simulink model "model"  (R2014a)
(part 4 of 5)

      | %<Name>
  bus355 : powerlib/Measurements/Load Flow Bus  LConnTagsString=a  ID=bus355  Vbase=110000  Vref=1  Vangle=0  VLF=1  angleLF=0
      settings: AttributesFormatString=|
      | %<ID>
      | %<Vbase>V
      | %<VLF>pu
      | %<angleLF>deg.
      | %<Name>
  bus356 : powerlib/Measurements/Load Flow Bus  LConnTagsString=a  ID=bus356  Vbase=220000  Vref=1  Vangle=0  VLF=1  angleLF=0
      settings: AttributesFormatString=|
      | %<ID>
      | %<Vbase>V
      | %<VLF>pu
      | %<angleLF>deg.
      | %<Name>
  bus357 : powerlib/Measurements/Load Flow Bus  LConnTagsString=a  ID=bus357  Vbase=220000  Vref=1  Vangle=0  VLF=1  angleLF=0
      settings: AttributesFormatString=|
      | %<ID>
      | %<Vbase>V
      | %<VLF>pu
      | %<angleLF>deg.
      | %<Name>
  bus358 : powerlib/Measurements/Load Flow Bus  LConnTagsString=a  ID=bus358  Vbase=220000  Vref=1  Vangle=0  VLF=1  angleLF=0
      settings: AttributesFormatString=|
      | %<ID>
      | %<Vbase>V
      | %<VLF>pu
      | %<angleLF>deg.
      | %<Name>
  bus359 : powerlib/Measurements/Load Flow Bus  LConnTagsString=a  ID=bus359  Vbase=220000  Vref=1  Vangle=0  VLF=1  angleLF=0
      settings: AttributesFormatString=|
      | %<ID>
      | %<Vbase>V
      | %<VLF>pu
      | %<angleLF>deg.
      | %<Name>
  bus36 : powerlib/Measurements/Load Flow Bus  LConnTagsString=a  ID=bus36  Vbase=220000  Vref=1  Vangle=0  VLF=1  angleLF=0
      settings: AttributesFormatString=|
      | %<ID>
      | %<Vbase>V
      | %<VLF>pu
      | %<angleLF>deg.
      | %<Name>
  bus360 : powerlib/Measurements/Load Flow Bus  LConnTagsString=a  ID=bus360  Vbase=220000  Vref=1  Vangle=0  VLF=1  angleLF=0
      settings: AttributesFormatString=|
      | %<ID>
      | %<Vbase>V
      | %<VLF>pu
      | %<angleLF>deg.
      | %<Name>
  bus361 : powerlib/Measurements/Load Flow Bus  LConnTagsString=a  ID=bus361  Vbase=220000  Vref=1  Vangle=0  VLF=1  angleLF=0
      settings: AttributesFormatString=|
      | %<ID>
      | %<Vbase>V
      | %<VLF>pu
      | %<angleLF>deg.
      | %<Name>
  bus362 : powerlib/Measurements/Load Flow Bus  LConnTagsString=a  ID=bus362  Vbase=220000  Vref=1  Vangle=0  VLF=1  angleLF=0
      settings: AttributesFormatString=|
      | %<ID>
      | %<Vbase>V
      | %<VLF>pu
      | %<angleLF>deg.
      | %<Name>
  bus363 : powerlib/Measurements/Load Flow Bus  LConnTagsString=a  ID=bus363  Vbase=220000  Vref=1  Vangle=0  VLF=1  angleLF=0
      settings: AttributesFormatString=|
      | %<ID>
      | %<Vbase>V
      | %<VLF>pu
      | %<angleLF>deg.
      | %<Name>
  bus364 : powerlib/Measurements/Load Flow Bus  LConnTagsString=a  ID=bus364  Vbase=220000  Vref=1  Vangle=0  VLF=1  angleLF=0
      settings: AttributesFormatString=|
      | %<ID>
      | %<Vbase>V
      | %<VLF>pu
      | %<angleLF>deg.
      | %<Name>
  bus365 : powerlib/Measurements/Load Flow Bus  LConnTagsString=a  ID=bus365  Vbase=220000  Vref=1  Vangle=0  VLF=1  angleLF=0
      settings: AttributesFormatString=|
      | %<ID>
      | %<Vbase>V
      | %<VLF>pu
      | %<angleLF>deg.
      | %<Name>
  bus366 : powerlib/Measurements/Load Flow Bus  LConnTagsString=a  ID=bus366  Vbase=220000  Vref=1  Vangle=0  VLF=1  angleLF=0
      settings: AttributesFormatString=|
      | %<ID>
      | %<Vbase>V
      | %<VLF>pu
      | %<angleLF>deg.
      | %<Name>
  bus367 : powerlib/Measurements/Load Flow Bus  LConnTagsString=a  ID=bus367  Vbase=220000  Vref=1  Vangle=0  VLF=1  angleLF=0
      settings: AttributesFormatString=|
      | %<ID>
      | %<Vbase>V
      | %<VLF>pu
      | %<angleLF>deg.
      | %<Name>
  bus368 : powerlib/Measurements/Load Flow Bus  LConnTagsString=a  ID=bus368  Vbase=220000  Vref=1  Vangle=0  VLF=1  angleLF=0
      settings: AttributesFormatString=|
      | %<ID>
      | %<Vbase>V
      | %<VLF>pu
      | %<angleLF>deg.
      | %<Name>
  bus369 : powerlib/Measurements/Load Flow Bus  LConnTagsString=a  ID=bus369  Vbase=220000  Vref=1  Vangle=0  VLF=1  angleLF=0
      settings: AttributesFormatString=|
      | %<ID>
      | %<Vbase>V
      | %<VLF>pu
      | %<angleLF>deg.
      | %<Name>
  bus37 : powerlib/Measurements/Load Flow Bus  LConnTagsString=a  ID=bus37  Vbase=220000  Vref=1  Vangle=0  VLF=1  angleLF=0
      settings: AttributesFormatString=|
      | %<ID>
      | %<Vbase>V
      | %<VLF>pu
      | %<angleLF>deg.
      | %<Name>
  bus370 : powerlib/Measurements/Load Flow Bus  LConnTagsString=a  ID=bus370  Vbase=220000  Vref=1  Vangle=0  VLF=1  angleLF=0
      settings: AttributesFormatString=|
      | %<ID>
      | %<Vbase>V
      | %<VLF>pu
      | %<angleLF>deg.
      | %<Name>
  bus371 : powerlib/Measurements/Load Flow Bus  LConnTagsString=a  ID=bus371  Vbase=220000  Vref=1  Vangle=0  VLF=1  angleLF=0
      settings: AttributesFormatString=|
      | %<ID>
      | %<Vbase>V
      | %<VLF>pu
      | %<angleLF>deg.
      | %<Name>
  bus372 : powerlib/Measurements/Load Flow Bus  LConnTagsString=a  ID=bus372  Vbase=220000  Vref=1  Vangle=0  VLF=1  angleLF=0
      settings: AttributesFormatString=|
      | %<ID>
      | %<Vbase>V
      | %<VLF>pu
      | %<angleLF>deg.
      | %<Name>
  bus373 : powerlib/Measurements/Load Flow Bus  LConnTagsString=a  ID=bus373  Vbase=220000  Vref=1  Vangle=0  VLF=1  angleLF=0
      settings: AttributesFormatString=|
      | %<ID>
      | %<Vbase>V
      | %<VLF>pu
      | %<angleLF>deg.
      | %<Name>
  bus374 : powerlib/Measurements/Load Flow Bus  LConnTagsString=a  ID=bus374  Vbase=220000  Vref=1  Vangle=0  VLF=1  angleLF=0
      settings: AttributesFormatString=|
      | %<ID>
      | %<Vbase>V
      | %<VLF>pu
      | %<angleLF>deg.
      | %<Name>
  bus375 : powerlib/Measurements/Load Flow Bus  LConnTagsString=a  ID=bus375  Vbase=220000  Vref=1  Vangle=0  VLF=1  angleLF=0
      settings: AttributesFormatString=|
      | %<ID>
      | %<Vbase>V
      | %<VLF>pu
      | %<angleLF>deg.
      | %<Name>
  bus376 : powerlib/Measurements/Load Flow Bus  LConnTagsString=a  ID=bus376  Vbase=220000  Vref=1  Vangle=0  VLF=1  angleLF=0
      settings: AttributesFormatString=|
      | %<ID>
      | %<Vbase>V
      | %<VLF>pu
      | %<angleLF>deg.
      | %<Name>
  bus377 : powerlib/Measurements/Load Flow Bus  LConnTagsString=a  ID=bus377  Vbase=220000  Vref=1  Vangle=0  VLF=1  angleLF=0
      settings: AttributesFormatString=|
      | %<ID>
      | %<Vbase>V
      | %<VLF>pu
      | %<angleLF>deg.
      | %<Name>
  bus378 : powerlib/Measurements/Load Flow Bus  LConnTagsString=a  ID=bus378  Vbase=220000  Vref=1  Vangle=0  VLF=1  angleLF=0
      settings: AttributesFormatString=|
      | %<ID>
      | %<Vbase>V
      | %<VLF>pu
      | %<angleLF>deg.
      | %<Name>
  bus379 : powerlib/Measurements/Load Flow Bus  LConnTagsString=a  ID=bus379  Vbase=220000  Vref=1  Vangle=0  VLF=1  angleLF=0
      settings: AttributesFormatString=|
      | %<ID>
      | %<Vbase>V
      | %<VLF>pu
      | %<angleLF>deg.
      | %<Name>
  bus38 : powerlib/Measurements/Load Flow Bus  LConnTagsString=a  ID=bus38  Vbase=220000  Vref=1  Vangle=0  VLF=1  angleLF=0
      settings: AttributesFormatString=|
      | %<ID>
      | %<Vbase>V
      | %<VLF>pu
      | %<angleLF>deg.
      | %<Name>
  bus380 : powerlib/Measurements/Load Flow Bus  LConnTagsString=a  ID=bus380  Vbase=220000  Vref=1  Vangle=0  VLF=1  angleLF=0
      settings: AttributesFormatString=|
      | %<ID>
      | %<Vbase>V
      | %<VLF>pu
      | %<angleLF>deg.
      | %<Name>
  bus381 : powerlib/Measurements/Load Flow Bus  LConnTagsString=a  ID=bus381  Vbase=220000  Vref=1  Vangle=0  VLF=1  angleLF=0
      settings: AttributesFormatString=|
      | %<ID>
      | %<Vbase>V
      | %<VLF>pu
      | %<angleLF>deg.
      | %<Name>
  bus382 : powerlib/Measurements/Load Flow Bus  LConnTagsString=a  ID=bus382  Vbase=220000  Vref=1  Vangle=0  VLF=1  angleLF=0
      settings: AttributesFormatString=|
      | %<ID>
      | %<Vbase>V
      | %<VLF>pu
      | %<angleLF>deg.
      | %<Name>
  bus383 : powerlib/Measurements/Load Flow Bus  LConnTagsString=a  ID=bus383  Vbase=220000  Vref=1  Vangle=0  VLF=1  angleLF=0
      settings: AttributesFormatString=|
      | %<ID>
      | %<Vbase>V
      | %<VLF>pu
      | %<angleLF>deg.
      | %<Name>
  bus384 : powerlib/Measurements/Load Flow Bus  LConnTagsString=a  ID=bus384  Vbase=220000  Vref=1  Vangle=0  VLF=1  angleLF=0
      settings: AttributesFormatString=|
      | %<ID>
      | %<Vbase>V
      | %<VLF>pu
      | %<angleLF>deg.
      | %<Name>
  bus385 : powerlib/Measurements/Load Flow Bus  LConnTagsString=a  ID=bus385  Vbase=220000  Vref=1  Vangle=0  VLF=1  angleLF=0
      settings: AttributesFormatString=|
      | %<ID>
      | %<Vbase>V
      | %<VLF>pu
      | %<angleLF>deg.
      | %<Name>
  bus386 : powerlib/Measurements/Load Flow Bus  LConnTagsString=a  ID=bus386  Vbase=220000  Vref=1  Vangle=0  VLF=1  angleLF=0
      settings: AttributesFormatString=|
      | %<ID>
      | %<Vbase>V
      | %<VLF>pu
      | %<angleLF>deg.
      | %<Name>
  bus387 : powerlib/Measurements/Load Flow Bus  LConnTagsString=a  ID=bus387  Vbase=220000  Vref=1  Vangle=0  VLF=1  angleLF=0
      settings: AttributesFormatString=|
      | %<ID>
      | %<Vbase>V
      | %<VLF>pu
      | %<angleLF>deg.
      | %<Name>
  bus388 : powerlib/Measurements/Load Flow Bus  LConnTagsString=a  ID=bus388  Vbase=220000  Vref=1  Vangle=0  VLF=1  angleLF=0
      settings: AttributesFormatString=|
      | %<ID>
      | %<Vbase>V
      | %<VLF>pu
      | %<angleLF>deg.
      | %<Name>
  bus389 : powerlib/Measurements/Load Flow Bus  LConnTagsString=a  ID=bus389  Vbase=220000  Vref=1  Vangle=0  VLF=1  angleLF=0
      settings: AttributesFormatString=|
      | %<ID>
      | %<Vbase>V
      | %<VLF>pu
      | %<angleLF>deg.
      | %<Name>
  bus39 : powerlib/Measurements/Load Flow Bus  LConnTagsString=a  ID=bus39  Vbase=220000  Vref=1  Vangle=0  VLF=1  angleLF=0
      settings: AttributesFormatString=|
      | %<ID>
      | %<Vbase>V
      | %<VLF>pu
      | %<angleLF>deg.
      | %<Name>
  bus390 : powerlib/Measurements/Load Flow Bus  LConnTagsString=a  ID=bus390  Vbase=220000  Vref=1  Vangle=0  VLF=1  angleLF=0
      settings: AttributesFormatString=|
      | %<ID>
      | %<Vbase>V
      | %<VLF>pu
      | %<angleLF>deg.
      | %<Name>
  bus391 : powerlib/Measurements/Load Flow Bus  LConnTagsString=a  ID=bus391  Vbase=220000  Vref=1  Vangle=0  VLF=1  angleLF=0
      settings: AttributesFormatString=|
      | %<ID>
      | %<Vbase>V
      | %<VLF>pu
      | %<angleLF>deg.
      | %<Name>
  bus392 : powerlib/Measurements/Load Flow Bus  LConnTagsString=a  ID=bus392  Vbase=220000  Vref=1  Vangle=0  VLF=1  angleLF=0
      settings: AttributesFormatString=|
      | %<ID>
      | %<Vbase>V
      | %<VLF>pu
      | %<angleLF>deg.
      | %<Name>
  bus393 : powerlib/Measurements/Load Flow Bus  LConnTagsString=a  ID=bus393  Vbase=220000  Vref=1  Vangle=0  VLF=1  angleLF=0
      settings: AttributesFormatString=|
      | %<ID>
      | %<Vbase>V
      | %<VLF>pu
      | %<angleLF>deg.
      | %<Name>
  bus394 : powerlib/Measurements/Load Flow Bus  LConnTagsString=a  ID=bus394  Vbase=220000  Vref=1  Vangle=0  VLF=1  angleLF=0
      settings: AttributesFormatString=|
      | %<ID>
      | %<Vbase>V
      | %<VLF>pu
      | %<angleLF>deg.
      | %<Name>
  bus395 : powerlib/Measurements/Load Flow Bus  LConnTagsString=a  ID=bus395  Vbase=220000  Vref=1  Vangle=0  VLF=1  angleLF=0
      settings: AttributesFormatString=|
      | %<ID>
      | %<Vbase>V
      | %<VLF>pu
      | %<angleLF>deg.
      | %<Name>
  bus396 : powerlib/Measurements/Load Flow Bus  LConnTagsString=a  ID=bus396  Vbase=220000  Vref=1  Vangle=0  VLF=1  angleLF=0
      settings: AttributesFormatString=|
      | %<ID>
      | %<Vbase>V
      | %<VLF>pu
      | %<angleLF>deg.
      | %<Name>
  bus397 : powerlib/Measurements/Load Flow Bus  LConnTagsString=a  ID=bus397  Vbase=220000  Vref=1  Vangle=0  VLF=1  angleLF=0
      settings: AttributesFormatString=|
      | %<ID>
      | %<Vbase>V
      | %<VLF>pu
      | %<angleLF>deg.
      | %<Name>
  bus398 : powerlib/Measurements/Load Flow Bus  LConnTagsString=a  ID=bus398  Vbase=220000  Vref=1  Vangle=0  VLF=1  angleLF=0
      settings: AttributesFormatString=|
      | %<ID>
      | %<Vbase>V
      | %<VLF>pu
      | %<angleLF>deg.
      | %<Name>
  bus399 : powerlib/Measurements/Load Flow Bus  LConnTagsString=a  ID=bus399  Vbase=220000  Vref=1  Vangle=0  VLF=1  angleLF=0
      settings: AttributesFormatString=|
      | %<ID>
      | %<Vbase>V
      | %<VLF>pu
      | %<angleLF>deg.
      | %<Name>
  bus4 : powerlib/Measurements/Load Flow Bus  LConnTagsString=a  ID=bus4  Vbase=110000  Vref=1  Vangle=0  VLF=1  angleLF=0
      settings: AttributesFormatString=|
      | %<ID>
      | %<Vbase>V
      | %<VLF>pu
      | %<angleLF>deg.
      | %<Name>
  bus40 : powerlib/Measurements/Load Flow Bus  LConnTagsString=a  ID=bus40  Vbase=220000  Vref=1  Vangle=0  VLF=1  angleLF=0
      settings: AttributesFormatString=|
      | %<ID>
      | %<Vbase>V
      | %<VLF>pu
      | %<angleLF>deg.
      | %<Name>
  bus400 : powerlib/Measurements/Load Flow Bus  LConnTagsString=a  ID=bus400  Vbase=220000  Vref=1  Vangle=0  VLF=1  angleLF=0
      settings: AttributesFormatString=|
      | %<ID>
      | %<Vbase>V
      | %<VLF>pu
      | %<angleLF>deg.
      | %<Name>
  bus401 : powerlib/Measurements/Load Flow Bus  LConnTagsString=a  ID=bus401  Vbase=220000  Vref=1  Vangle=0  VLF=1  angleLF=0
      settings: AttributesFormatString=|
      | %<ID>
      | %<Vbase>V
      | %<VLF>pu
      | %<angleLF>deg.
      | %<Name>
  bus402 : powerlib/Measurements/Load Flow Bus  LConnTagsString=a  ID=bus402  Vbase=220000  Vref=1  Vangle=0  VLF=1  angleLF=0
      settings: AttributesFormatString=|
      | %<ID>
      | %<Vbase>V
      | %<VLF>pu
      | %<angleLF>deg.
      | %<Name>
  bus403 : powerlib/Measurements/Load Flow Bus  LConnTagsString=a  ID=bus403  Vbase=220000  Vref=1  Vangle=0  VLF=1  angleLF=0
      settings: AttributesFormatString=|
      | %<ID>
      | %<Vbase>V
      | %<VLF>pu
      | %<angleLF>deg.
      | %<Name>
  bus404 : powerlib/Measurements/Load Flow Bus  LConnTagsString=a  ID=bus404  Vbase=220000  Vref=1  Vangle=0  VLF=1  angleLF=0
      settings: AttributesFormatString=|
      | %<ID>
      | %<Vbase>V
      | %<VLF>pu
      | %<angleLF>deg.
      | %<Name>
  bus405 : powerlib/Measurements/Load Flow Bus  LConnTagsString=a  ID=bus405  Vbase=220000  Vref=1  Vangle=0  VLF=1  angleLF=0
      settings: AttributesFormatString=|
      | %<ID>
      | %<Vbase>V
      | %<VLF>pu
      | %<angleLF>deg.
      | %<Name>
  bus406 : powerlib/Measurements/Load Flow Bus  LConnTagsString=a  ID=bus406  Vbase=220000  Vref=1  Vangle=0  VLF=1  angleLF=0
      settings: AttributesFormatString=|
      | %<ID>
      | %<Vbase>V
      | %<VLF>pu
      | %<angleLF>deg.
      | %<Name>
  bus407 : powerlib/Measurements/Load Flow Bus  LConnTagsString=a  ID=bus407  Vbase=220000  Vref=1  Vangle=0  VLF=1  angleLF=0
      settings: AttributesFormatString=|
      | %<ID>
      | %<Vbase>V
      | %<VLF>pu
      | %<angleLF>deg.
      | %<Name>
  bus408 : powerlib/Measurements/Load Flow Bus  LConnTagsString=a  ID=bus408  Vbase=220000  Vref=1  Vangle=0  VLF=1  angleLF=0
      settings: AttributesFormatString=|
      | %<ID>
      | %<Vbase>V
      | %<VLF>pu
      | %<angleLF>deg.
      | %<Name>
  bus409 : powerlib/Measurements/Load Flow Bus  LConnTagsString=a  ID=bus409  Vbase=220000  Vref=1  Vangle=0  VLF=1  angleLF=0
      settings: AttributesFormatString=|
      | %<ID>
      | %<Vbase>V
      | %<VLF>pu
      | %<angleLF>deg.
      | %<Name>
  bus41 : powerlib/Measurements/Load Flow Bus  LConnTagsString=a  ID=bus41  Vbase=220000  Vref=1  Vangle=0  VLF=1  angleLF=0
      settings: AttributesFormatString=|
      | %<ID>
      | %<Vbase>V
      | %<VLF>pu
      | %<angleLF>deg.
      | %<Name>
  bus410 : powerlib/Measurements/Load Flow Bus  LConnTagsString=a  ID=bus410  Vbase=220000  Vref=1  Vangle=0  VLF=1  angleLF=0
      settings: AttributesFormatString=|
      | %<ID>
      | %<Vbase>V
      | %<VLF>pu
      | %<angleLF>deg.
      | %<Name>
  bus411 : powerlib/Measurements/Load Flow Bus  LConnTagsString=a  ID=bus411  Vbase=220000  Vref=1  Vangle=0  VLF=1  angleLF=0
      settings: AttributesFormatString=|
      | %<ID>
      | %<Vbase>V
      | %<VLF>pu
      | %<angleLF>deg.
      | %<Name>
  bus412 : powerlib/Measurements/Load Flow Bus  LConnTagsString=a  ID=bus412  Vbase=220000  Vref=1  Vangle=0  VLF=1  angleLF=0
      settings: AttributesFormatString=|
      | %<ID>
      | %<Vbase>V
      | %<VLF>pu
      | %<angleLF>deg.
      | %<Name>
  bus413 : powerlib/Measurements/Load Flow Bus  LConnTagsString=a  ID=bus413  Vbase=220000  Vref=1  Vangle=0  VLF=1  angleLF=0
      settings: AttributesFormatString=|
      | %<ID>
      | %<Vbase>V
      | %<VLF>pu
      | %<angleLF>deg.
      | %<Name>
  bus414 : powerlib/Measurements/Load Flow Bus  LConnTagsString=a  ID=bus414  Vbase=220000  Vref=1  Vangle=0  VLF=1  angleLF=0
      settings: AttributesFormatString=|
      | %<ID>
      | %<Vbase>V
      | %<VLF>pu
      | %<angleLF>deg.
      | %<Name>
  bus415 : powerlib/Measurements/Load Flow Bus  LConnTagsString=a  ID=bus415  Vbase=220000  Vref=1  Vangle=0  VLF=1  angleLF=0
      settings: AttributesFormatString=|
      | %<ID>
      | %<Vbase>V
      | %<VLF>pu
      | %<angleLF>deg.
      | %<Name>
  bus416 : powerlib/Measurements/Load Flow Bus  LConnTagsString=a  ID=bus416  Vbase=220000  Vref=1  Vangle=0  VLF=1  angleLF=0
      settings: AttributesFormatString=|
      | %<ID>
      | %<Vbase>V
      | %<VLF>pu
      | %<angleLF>deg.
      | %<Name>
  bus417 : powerlib/Measurements/Load Flow Bus  LConnTagsString=a  ID=bus417  Vbase=220000  Vref=1  Vangle=0  VLF=1  angleLF=0
      settings: AttributesFormatString=|
      | %<ID>
      | %<Vbase>V
      | %<VLF>pu
      | %<angleLF>deg.
      | %<Name>
  bus418 : powerlib/Measurements/Load Flow Bus  LConnTagsString=a  ID=bus418  Vbase=220000  Vref=1  Vangle=0  VLF=1  angleLF=0
      settings: AttributesFormatString=|
      | %<ID>
      | %<Vbase>V
      | %<VLF>pu
      | %<angleLF>deg.
      | %<Name>
  bus419 : powerlib/Measurements/Load Flow Bus  LConnTagsString=a  ID=bus419  Vbase=220000  Vref=1  Vangle=0  VLF=1  angleLF=0
      settings: AttributesFormatString=|
      | %<ID>
      | %<Vbase>V
      | %<VLF>pu
      | %<angleLF>deg.
      | %<Name>
  bus42 : powerlib/Measurements/Load Flow Bus  LConnTagsString=a  ID=bus42  Vbase=220000  Vref=1  Vangle=0  VLF=1  angleLF=0
      settings: AttributesFormatString=|
      | %<ID>
      | %<Vbase>V
      | %<VLF>pu
      | %<angleLF>deg.
      | %<Name>
  bus420 : powerlib/Measurements/Load Flow Bus  LConnTagsString=a  ID=bus420  Vbase=220000  Vref=1  Vangle=0  VLF=1  angleLF=0
      settings: AttributesFormatString=|
      | %<ID>
      | %<Vbase>V
      | %<VLF>pu
      | %<angleLF>deg.
      | %<Name>
  bus421 : powerlib/Measurements/Load Flow Bus  LConnTagsString=a  ID=bus421  Vbase=220000  Vref=1  Vangle=0  VLF=1  angleLF=0
      settings: AttributesFormatString=|
      | %<ID>
      | %<Vbase>V
      | %<VLF>pu
      | %<angleLF>deg.
      | %<Name>
  bus422 : powerlib/Measurements/Load Flow Bus  LConnTagsString=a  ID=bus422  Vbase=220000  Vref=1  Vangle=0  VLF=1  angleLF=0
      settings: AttributesFormatString=|
      | %<ID>
      | %<Vbase>V
      | %<VLF>pu
      | %<angleLF>deg.
      | %<Name>
  bus423 : powerlib/Measurements/Load Flow Bus  LConnTagsString=a  ID=bus423  Vbase=220000  Vref=1  Vangle=0  VLF=1  angleLF=0
      settings: AttributesFormatString=|
      | %<ID>
      | %<Vbase>V
      | %<VLF>pu
      | %<angleLF>deg.
      | %<Name>
  bus424 : powerlib/Measurements/Load Flow Bus  LConnTagsString=a  ID=bus424  Vbase=220000  Vref=1  Vangle=0  VLF=1  angleLF=0
      settings: AttributesFormatString=|
      | %<ID>
      | %<Vbase>V
      | %<VLF>pu
      | %<angleLF>deg.
      | %<Name>
  bus425 : powerlib/Measurements/Load Flow Bus  LConnTagsString=a  ID=bus425  Vbase=220000  Vref=1  Vangle=0  VLF=1  angleLF=0
      settings: AttributesFormatString=|
      | %<ID>
      | %<Vbase>V
      | %<VLF>pu
      | %<angleLF>deg.
      | %<Name>
  bus426 : powerlib/Measurements/Load Flow Bus  LConnTagsString=a  ID=bus426  Vbase=220000  Vref=1  Vangle=0  VLF=1  angleLF=0
      settings: AttributesFormatString=|
      | %<ID>
      | %<Vbase>V
      | %<VLF>pu
      | %<angleLF>deg.
      | %<Name>
  bus427 : powerlib/Measurements/Load Flow Bus  LConnTagsString=a  ID=bus427  Vbase=220000  Vref=1  Vangle=0  VLF=1  angleLF=0
      settings: AttributesFormatString=|
      | %<ID>
      | %<Vbase>V
      | %<VLF>pu
      | %<angleLF>deg.
      | %<Name>
  bus428 : powerlib/Measurements/Load Flow Bus  LConnTagsString=a  ID=bus428  Vbase=220000  Vref=1  Vangle=0  VLF=1  angleLF=0
      settings: AttributesFormatString=|
      | %<ID>
      | %<Vbase>V
      | %<VLF>pu
      | %<angleLF>deg.
      | %<Name>
  bus429 : powerlib/Measurements/Load Flow Bus  LConnTagsString=a  ID=bus429  Vbase=220000  Vref=1  Vangle=0  VLF=1  angleLF=0
      settings: AttributesFormatString=|
      | %<ID>
      | %<Vbase>V
      | %<VLF>pu
      | %<angleLF>deg.
      | %<Name>
  bus43 : powerlib/Measurements/Load Flow Bus  LConnTagsString=a  ID=bus43  Vbase=220000  Vref=1  Vangle=0  VLF=1  angleLF=0
      settings: AttributesFormatString=|
      | %<ID>
      | %<Vbase>V
      | %<VLF>pu
      | %<angleLF>deg.
      | %<Name>
  bus430 : powerlib/Measurements/Load Flow Bus  LConnTagsString=a  ID=bus430  Vbase=220000  Vref=1  Vangle=0  VLF=1  angleLF=0
      settings: AttributesFormatString=|
      | %<ID>
      | %<Vbase>V
      | %<VLF>pu
      | %<angleLF>deg.
      | %<Name>
  bus431 : powerlib/Measurements/Load Flow Bus  LConnTagsString=a  ID=bus431  Vbase=220000  Vref=1  Vangle=0  VLF=1  angleLF=0
      settings: AttributesFormatString=|
      | %<ID>
      | %<Vbase>V
      | %<VLF>pu
      | %<angleLF>deg.
      | %<Name>
  bus432 : powerlib/Measurements/Load Flow Bus  LConnTagsString=a  ID=bus432  Vbase=220000  Vref=1  Vangle=0  VLF=1  angleLF=0
      settings: AttributesFormatString=|
      | %<ID>
      | %<Vbase>V
      | %<VLF>pu
      | %<angleLF>deg.
      | %<Name>
  bus433 : powerlib/Measurements/Load Flow Bus  LConnTagsString=a  ID=bus433  Vbase=220000  Vref=1  Vangle=0  VLF=1  angleLF=0
      settings: AttributesFormatString=|
      | %<ID>
      | %<Vbase>V
      | %<VLF>pu
      | %<angleLF>deg.
      | %<Name>
  bus434 : powerlib/Measurements/Load Flow Bus  LConnTagsString=a  ID=bus434  Vbase=220000  Vref=1  Vangle=0  VLF=1  angleLF=0
      settings: AttributesFormatString=|
      | %<ID>
      | %<Vbase>V
      | %<VLF>pu
      | %<angleLF>deg.
      | %<Name>
  bus435 : powerlib/Measurements/Load Flow Bus  LConnTagsString=a  ID=bus435  Vbase=220000  Vref=1  Vangle=0  VLF=1  angleLF=0
      settings: AttributesFormatString=|
      | %<ID>
      | %<Vbase>V
      | %<VLF>pu
      | %<angleLF>deg.
      | %<Name>
  bus436 : powerlib/Measurements/Load Flow Bus  LConnTagsString=a  ID=bus436  Vbase=220000  Vref=1  Vangle=0  VLF=1  angleLF=0
      settings: AttributesFormatString=|
      | %<ID>
      | %<Vbase>V
      | %<VLF>pu
      | %<angleLF>deg.
      | %<Name>
  bus437 : powerlib/Measurements/Load Flow Bus  LConnTagsString=a  ID=bus437  Vbase=220000  Vref=1  Vangle=0  VLF=1  angleLF=0
      settings: AttributesFormatString=|
      | %<ID>
      | %<Vbase>V
      | %<VLF>pu
      | %<angleLF>deg.
      | %<Name>
  bus438 : powerlib/Measurements/Load Flow Bus  LConnTagsString=a  ID=bus438  Vbase=220000  Vref=1  Vangle=0  VLF=1  angleLF=0
      settings: AttributesFormatString=|
      | %<ID>
      | %<Vbase>V
      | %<VLF>pu
      | %<angleLF>deg.
      | %<Name>
  bus439 : powerlib/Measurements/Load Flow Bus  LConnTagsString=a  ID=bus439  Vbase=220000  Vref=1  Vangle=0  VLF=1  angleLF=0
      settings: AttributesFormatString=|
      | %<ID>
      | %<Vbase>V
      | %<VLF>pu
      | %<angleLF>deg.
      | %<Name>
  bus44 : powerlib/Measurements/Load Flow Bus  LConnTagsString=a  ID=bus44  Vbase=220000  Vref=1  Vangle=0  VLF=1  angleLF=0
      settings: AttributesFormatString=|
      | %<ID>
      | %<Vbase>V
      | %<VLF>pu
      | %<angleLF>deg.
      | %<Name>
  bus440 : powerlib/Measurements/Load Flow Bus  LConnTagsString=a  ID=bus440  Vbase=220000  Vref=1  Vangle=0  VLF=1  angleLF=0
      settings: AttributesFormatString=|
      | %<ID>
      | %<Vbase>V
      | %<VLF>pu
      | %<angleLF>deg.
      | %<Name>
  bus441 : powerlib/Measurements/Load Flow Bus  LConnTagsString=a  ID=bus441  Vbase=220000  Vref=1  Vangle=0  VLF=1  angleLF=0
      settings: AttributesFormatString=|
      | %<ID>
      | %<Vbase>V
      | %<VLF>pu
      | %<angleLF>deg.
      | %<Name>
  bus442 : powerlib/Measurements/Load Flow Bus  LConnTagsString=a  ID=bus442  Vbase=220000  Vref=1  Vangle=0  VLF=1  angleLF=0
      settings: AttributesFormatString=|
      | %<ID>
      | %<Vbase>V
      | %<VLF>pu
      | %<angleLF>deg.
      | %<Name>
  bus443 : powerlib/Measurements/Load Flow Bus  LConnTagsString=a  ID=bus443  Vbase=220000  Vref=1  Vangle=0  VLF=1  angleLF=0
      settings: AttributesFormatString=|
      | %<ID>
      | %<Vbase>V
      | %<VLF>pu
      | %<angleLF>deg.
      | %<Name>
  bus444 : powerlib/Measurements/Load Flow Bus  LConnTagsString=a  ID=bus444  Vbase=220000  Vref=1  Vangle=0  VLF=1  angleLF=0
      settings: AttributesFormatString=|
      | %<ID>
      | %<Vbase>V
      | %<VLF>pu
      | %<angleLF>deg.
      | %<Name>
  bus445 : powerlib/Measurements/Load Flow Bus  LConnTagsString=a  ID=bus445  Vbase=220000  Vref=1  Vangle=0  VLF=1  angleLF=0
      settings: AttributesFormatString=|
      | %<ID>
      | %<Vbase>V
      | %<VLF>pu
      | %<angleLF>deg.
      | %<Name>
  bus446 : powerlib/Measurements/Load Flow Bus  LConnTagsString=a  ID=bus446  Vbase=220000  Vref=1  Vangle=0  VLF=1  angleLF=0
      settings: AttributesFormatString=|
      | %<ID>
      | %<Vbase>V
      | %<VLF>pu
      | %<angleLF>deg.
      | %<Name>
  bus447 : powerlib/Measurements/Load Flow Bus  LConnTagsString=a  ID=bus447  Vbase=220000  Vref=1  Vangle=0  VLF=1  angleLF=0
      settings: AttributesFormatString=|
      | %<ID>
      | %<Vbase>V
      | %<VLF>pu
      | %<angleLF>deg.
      | %<Name>
  bus448 : powerlib/Measurements/Load Flow Bus  LConnTagsString=a  ID=bus448  Vbase=220000  Vref=1  Vangle=0  VLF=1  angleLF=0
      settings: AttributesFormatString=|
      | %<ID>
      | %<Vbase>V
      | %<VLF>pu
      | %<angleLF>deg.
      | %<Name>
  bus449 : powerlib/Measurements/Load Flow Bus  LConnTagsString=a  ID=bus449  Vbase=220000  Vref=1  Vangle=0  VLF=1  angleLF=0
      settings: AttributesFormatString=|
      | %<ID>
      | %<Vbase>V
      | %<VLF>pu
      | %<angleLF>deg.
      | %<Name>
  bus45 : powerlib/Measurements/Load Flow Bus  LConnTagsString=a  ID=bus45  Vbase=220000  Vref=1  Vangle=0  VLF=1  angleLF=0
      settings: AttributesFormatString=|
      | %<ID>
      | %<Vbase>V
      | %<VLF>pu
      | %<angleLF>deg.
      | %<Name>
  bus450 : powerlib/Measurements/Load Flow Bus  LConnTagsString=a  ID=bus450  Vbase=220000  Vref=1  Vangle=0  VLF=1  angleLF=0
      settings: AttributesFormatString=|
      | %<ID>
      | %<Vbase>V
      | %<VLF>pu
      | %<angleLF>deg.
      | %<Name>
  bus451 : powerlib/Measurements/Load Flow Bus  LConnTagsString=a  ID=bus451  Vbase=220000  Vref=1  Vangle=0  VLF=1  angleLF=0
      settings: AttributesFormatString=|
      | %<ID>
      | %<Vbase>V
      | %<VLF>pu
      | %<angleLF>deg.
      | %<Name>
  bus452 : powerlib/Measurements/Load Flow Bus  LConnTagsString=a  ID=bus452  Vbase=220000  Vref=1  Vangle=0  VLF=1  angleLF=0
      settings: AttributesFormatString=|
      | %<ID>
      | %<Vbase>V
      | %<VLF>pu
      | %<angleLF>deg.
      | %<Name>
  bus453 : powerlib/Measurements/Load Flow Bus  LConnTagsString=a  ID=bus453  Vbase=220000  Vref=1  Vangle=0  VLF=1  angleLF=0
      settings: AttributesFormatString=|
      | %<ID>
      | %<Vbase>V
      | %<VLF>pu
      | %<angleLF>deg.
      | %<Name>
  bus454 : powerlib/Measurements/Load Flow Bus  LConnTagsString=a  ID=bus454  Vbase=220000  Vref=1  Vangle=0  VLF=1  angleLF=0
      settings: AttributesFormatString=|
      | %<ID>
      | %<Vbase>V
      | %<VLF>pu
      | %<angleLF>deg.
      | %<Name>
  bus455 : powerlib/Measurements/Load Flow Bus  LConnTagsString=a  ID=bus455  Vbase=220000  Vref=1  Vangle=0  VLF=1  angleLF=0
      settings: AttributesFormatString=|
      | %<ID>
      | %<Vbase>V
      | %<VLF>pu
      | %<angleLF>deg.
      | %<Name>
  bus456 : powerlib/Measurements/Load Flow Bus  LConnTagsString=a  ID=bus456  Vbase=220000  Vref=1  Vangle=0  VLF=1  angleLF=0
      settings: AttributesFormatString=|
      | %<ID>
      | %<Vbase>V
      | %<VLF>pu
      | %<angleLF>deg.
      | %<Name>
  bus457 : powerlib/Measurements/Load Flow Bus  LConnTagsString=a  ID=bus457  Vbase=220000  Vref=1  Vangle=0  VLF=1  angleLF=0
      settings: AttributesFormatString=|
      | %<ID>
      | %<Vbase>V
      | %<VLF>pu
      | %<angleLF>deg.
      | %<Name>
  bus458 : powerlib/Measurements/Load Flow Bus  LConnTagsString=a  ID=bus458  Vbase=220000  Vref=1  Vangle=0  VLF=1  angleLF=0
      settings: AttributesFormatString=|
      | %<ID>
      | %<Vbase>V
      | %<VLF>pu
      | %<angleLF>deg.
      | %<Name>
  bus459 : powerlib/Measurements/Load Flow Bus  LConnTagsString=a  ID=bus459  Vbase=220000  Vref=1  Vangle=0  VLF=1  angleLF=0
      settings: AttributesFormatString=|
      | %<ID>
      | %<Vbase>V
      | %<VLF>pu
      | %<angleLF>deg.
      | %<Name>
  bus46 : powerlib/Measurements/Load Flow Bus  LConnTagsString=a  ID=bus46  Vbase=220000  Vref=1  Vangle=0  VLF=1  angleLF=0
      settings: AttributesFormatString=|
      | %<ID>
      | %<Vbase>V
      | %<VLF>pu
      | %<angleLF>deg.
      | %<Name>
  bus460 : powerlib/Measurements/Load Flow Bus  LConnTagsString=a  ID=bus460  Vbase=220000  Vref=1  Vangle=0  VLF=1  angleLF=0
      settings: AttributesFormatString=|
      | %<ID>
      | %<Vbase>V
      | %<VLF>pu
      | %<angleLF>deg.
      | %<Name>
  bus461 : powerlib/Measurements/Load Flow Bus  LConnTagsString=a  ID=bus461  Vbase=220000  Vref=1  Vangle=0  VLF=1  angleLF=0
      settings: AttributesFormatString=|
      | %<ID>
      | %<Vbase>V
      | %<VLF>pu
      | %<angleLF>deg.
      | %<Name>
  bus462 : powerlib/Measurements/Load Flow Bus  LConnTagsString=a  ID=bus462  Vbase=220000  Vref=1  Vangle=0  VLF=1  angleLF=0
      settings: AttributesFormatString=|
      | %<ID>
      | %<Vbase>V
      | %<VLF>pu
      | %<angleLF>deg.
      | %<Name>
  bus463 : powerlib/Measurements/Load Flow Bus  LConnTagsString=a  ID=bus463  Vbase=220000  Vref=1  Vangle=0  VLF=1  angleLF=0
      settings: AttributesFormatString=|
      | %<ID>
      | %<Vbase>V
      | %<VLF>pu
      | %<angleLF>deg.
      | %<Name>
  bus464 : powerlib/Measurements/Load Flow Bus  LConnTagsString=a  ID=bus464  Vbase=220000  Vref=1  Vangle=0  VLF=1  angleLF=0
      settings: AttributesFormatString=|
      | %<ID>
      | %<Vbase>V
      | %<VLF>pu
      | %<angleLF>deg.
      | %<Name>
  bus465 : powerlib/Measurements/Load Flow Bus  LConnTagsString=a  ID=bus465  Vbase=220000  Vref=1  Vangle=0  VLF=1  angleLF=0
      settings: AttributesFormatString=|
      | %<ID>
      | %<Vbase>V
      | %<VLF>pu
      | %<angleLF>deg.
      | %<Name>
  bus466 : powerlib/Measurements/Load Flow Bus  LConnTagsString=a  ID=bus466  Vbase=220000  Vref=1  Vangle=0  VLF=1  angleLF=0
      settings: AttributesFormatString=|
      | %<ID>
      | %<Vbase>V
      | %<VLF>pu
      | %<angleLF>deg.
      | %<Name>
  bus467 : powerlib/Measurements/Load Flow Bus  LConnTagsString=a  ID=bus467  Vbase=220000  Vref=1  Vangle=0  VLF=1  angleLF=0
      settings: AttributesFormatString=|
      | %<ID>
      | %<Vbase>V
      | %<VLF>pu
      | %<angleLF>deg.
      | %<Name>
  bus468 : powerlib/Measurements/Load Flow Bus  LConnTagsString=a  ID=bus468  Vbase=220000  Vref=1  Vangle=0  VLF=1  angleLF=0
      settings: AttributesFormatString=|
      | %<ID>
      | %<Vbase>V
      | %<VLF>pu
      | %<angleLF>deg.
      | %<Name>
  bus469 : powerlib/Measurements/Load Flow Bus  LConnTagsString=a  ID=bus469  Vbase=220000  Vref=1  Vangle=0  VLF=1  angleLF=0
      settings: AttributesFormatString=|
      | %<ID>
      | %<Vbase>V
      | %<VLF>pu
      | %<angleLF>deg.
      | %<Name>
  bus47 : powerlib/Measurements/Load Flow Bus  LConnTagsString=a  ID=bus47  Vbase=220000  Vref=1  Vangle=0  VLF=1  angleLF=0
      settings: AttributesFormatString=|
      | %<ID>
      | %<Vbase>V
      | %<VLF>pu
      | %<angleLF>deg.
      | %<Name>
  bus470 : powerlib/Measurements/Load Flow Bus  LConnTagsString=a  ID=bus470  Vbase=220000  Vref=1  Vangle=0  VLF=1  angleLF=0
      settings: AttributesFormatString=|
      | %<ID>
      | %<Vbase>V
      | %<VLF>pu
      | %<angleLF>deg.
      | %<Name>
  bus471 : powerlib/Measurements/Load Flow Bus  LConnTagsString=a  ID=bus471  Vbase=220000  Vref=1  Vangle=0  VLF=1  angleLF=0
      settings: AttributesFormatString=|
      | %<ID>
      | %<Vbase>V
      | %<VLF>pu
      | %<angleLF>deg.
      | %<Name>
  bus472 : powerlib/Measurements/Load Flow Bus  LConnTagsString=a  ID=bus472  Vbase=220000  Vref=1  Vangle=0  VLF=1  angleLF=0
      settings: AttributesFormatString=|
      | %<ID>
      | %<Vbase>V
      | %<VLF>pu
      | %<angleLF>deg.
      | %<Name>
  bus473 : powerlib/Measurements/Load Flow Bus  LConnTagsString=a  ID=bus473  Vbase=220000  Vref=1  Vangle=0  VLF=1  angleLF=0
      settings: AttributesFormatString=|
      | %<ID>
      | %<Vbase>V
      | %<VLF>pu
      | %<angleLF>deg.
      | %<Name>
  bus474 : powerlib/Measurements/Load Flow Bus  LConnTagsString=a  ID=bus474  Vbase=220000  Vref=1  Vangle=0  VLF=1  angleLF=0
      settings: AttributesFormatString=|
      | %<ID>
      | %<Vbase>V
      | %<VLF>pu
      | %<angleLF>deg.
      | %<Name>
  bus475 : powerlib/Measurements/Load Flow Bus  LConnTagsString=a  ID=bus475  Vbase=220000  Vref=1  Vangle=0  VLF=1  angleLF=0
      settings: AttributesFormatString=|
      | %<ID>
      | %<Vbase>V
      | %<VLF>pu
      | %<angleLF>deg.
      | %<Name>
  bus476 : powerlib/Measurements/Load Flow Bus  LConnTagsString=a  ID=bus476  Vbase=220000  Vref=1  Vangle=0  VLF=1  angleLF=0
      settings: AttributesFormatString=|
      | %<ID>
      | %<Vbase>V
      | %<VLF>pu
      | %<angleLF>deg.
      | %<Name>
  bus477 : powerlib/Measurements/Load Flow Bus  LConnTagsString=a  ID=bus477  Vbase=220000  Vref=1  Vangle=0  VLF=1  angleLF=0
      settings: AttributesFormatString=|
      | %<ID>
      | %<Vbase>V
      | %<VLF>pu
      | %<angleLF>deg.
      | %<Name>
  bus478 : powerlib/Measurements/Load Flow Bus  LConnTagsString=a  ID=bus478  Vbase=220000  Vref=1  Vangle=0  VLF=1  angleLF=0
      settings: AttributesFormatString=|
      | %<ID>
      | %<Vbase>V
      | %<VLF>pu
      | %<angleLF>deg.
      | %<Name>
  bus479 : powerlib/Measurements/Load Flow Bus  LConnTagsString=a  ID=bus479  Vbase=220000  Vref=1  Vangle=0  VLF=1  angleLF=0
      settings: AttributesFormatString=|
      | %<ID>
      | %<Vbase>V
      | %<VLF>pu
      | %<angleLF>deg.
      | %<Name>
  bus48 : powerlib/Measurements/Load Flow Bus  LConnTagsString=a  ID=bus48  Vbase=220000  Vref=1  Vangle=0  VLF=1  angleLF=0
      settings: AttributesFormatString=|
      | %<ID>
      | %<Vbase>V
      | %<VLF>pu
      | %<angleLF>deg.
      | %<Name>
  bus480 : powerlib/Measurements/Load Flow Bus  LConnTagsString=a  ID=bus480  Vbase=220000  Vref=1  Vangle=0  VLF=1  angleLF=0
      settings: AttributesFormatString=|
      | %<ID>
      | %<Vbase>V
      | %<VLF>pu
      | %<angleLF>deg.
      | %<Name>
  bus481 : powerlib/Measurements/Load Flow Bus  LConnTagsString=a  ID=bus481  Vbase=220000  Vref=1  Vangle=0  VLF=1  angleLF=0
      settings: AttributesFormatString=|
      | %<ID>
      | %<Vbase>V
      | %<VLF>pu
      | %<angleLF>deg.
      | %<Name>
  bus482 : powerlib/Measurements/Load Flow Bus  LConnTagsString=a  ID=bus482  Vbase=220000  Vref=1  Vangle=0  VLF=1  angleLF=0
      settings: AttributesFormatString=|
      | %<ID>
      | %<Vbase>V
      | %<VLF>pu
      | %<angleLF>deg.
      | %<Name>
  bus483 : powerlib/Measurements/Load Flow Bus  LConnTagsString=a  ID=bus483  Vbase=220000  Vref=1  Vangle=0  VLF=1  angleLF=0
      settings: AttributesFormatString=|
      | %<ID>
      | %<Vbase>V
      | %<VLF>pu
      | %<angleLF>deg.
      | %<Name>
  bus484 : powerlib/Measurements/Load Flow Bus  LConnTagsString=a  ID=bus484  Vbase=220000  Vref=1  Vangle=0  VLF=1  angleLF=0
      settings: AttributesFormatString=|
      | %<ID>
      | %<Vbase>V
      | %<VLF>pu
      | %<angleLF>deg.
      | %<Name>
  bus485 : powerlib/Measurements/Load Flow Bus  LConnTagsString=a  ID=bus485  Vbase=220000  Vref=1  Vangle=0  VLF=1  angleLF=0
      settings: AttributesFormatString=|
      | %<ID>
      | %<Vbase>V
      | %<VLF>pu
      | %<angleLF>deg.
      | %<Name>
  bus486 : powerlib/Measurements/Load Flow Bus  LConnTagsString=a  ID=bus486  Vbase=220000  Vref=1  Vangle=0  VLF=1  angleLF=0
      settings: AttributesFormatString=|
      | %<ID>
      | %<Vbase>V
      | %<VLF>pu
      | %<angleLF>deg.
      | %<Name>
  bus487 : powerlib/Measurements/Load Flow Bus  LConnTagsString=a  ID=bus487  Vbase=220000  Vref=1  Vangle=0  VLF=1  angleLF=0
      settings: AttributesFormatString=|
      | %<ID>
      | %<Vbase>V
      | %<VLF>pu
      | %<angleLF>deg.
      | %<Name>
  bus488 : powerlib/Measurements/Load Flow Bus  LConnTagsString=a  ID=bus488  Vbase=220000  Vref=1  Vangle=0  VLF=1  angleLF=0
      settings: AttributesFormatString=|
      | %<ID>
      | %<Vbase>V
      | %<VLF>pu
      | %<angleLF>deg.
      | %<Name>
  bus489 : powerlib/Measurements/Load Flow Bus  LConnTagsString=a  ID=bus489  Vbase=220000  Vref=1  Vangle=0  VLF=1  angleLF=0
      settings: AttributesFormatString=|
      | %<ID>
      | %<Vbase>V
      | %<VLF>pu
      | %<angleLF>deg.
      | %<Name>
  bus49 : powerlib/Measurements/Load Flow Bus  LConnTagsString=a  ID=bus49  Vbase=220000  Vref=1  Vangle=0  VLF=1  angleLF=0
      settings: AttributesFormatString=|
      | %<ID>
      | %<Vbase>V
      | %<VLF>pu
      | %<angleLF>deg.
      | %<Name>
  bus490 : powerlib/Measurements/Load Flow Bus  LConnTagsString=a  ID=bus490  Vbase=220000  Vref=1  Vangle=0  VLF=1  angleLF=0
      settings: AttributesFormatString=|
      | %<ID>
      | %<Vbase>V
      | %<VLF>pu
      | %<angleLF>deg.
      | %<Name>
  bus491 : powerlib/Measurements/Load Flow Bus  LConnTagsString=a  ID=bus491  Vbase=220000  Vref=1  Vangle=0  VLF=1  angleLF=0
      settings: AttributesFormatString=|
      | %<ID>
      | %<Vbase>V
      | %<VLF>pu
      | %<angleLF>deg.
      | %<Name>
  bus492 : powerlib/Measurements/Load Flow Bus  LConnTagsString=a  ID=bus492  Vbase=220000  Vref=1  Vangle=0  VLF=1  angleLF=0
      settings: AttributesFormatString=|
      | %<ID>
      | %<Vbase>V
      | %<VLF>pu
      | %<angleLF>deg.
      | %<Name>
  bus493 : powerlib/Measurements/Load Flow Bus  LConnTagsString=a  ID=bus493  Vbase=220000  Vref=1  Vangle=0  VLF=1  angleLF=0
      settings: AttributesFormatString=|
      | %<ID>
      | %<Vbase>V
      | %<VLF>pu
      | %<angleLF>deg.
      | %<Name>
  bus494 : powerlib/Measurements/Load Flow Bus  LConnTagsString=a  ID=bus494  Vbase=220000  Vref=1  Vangle=0  VLF=1  angleLF=0
      settings: AttributesFormatString=|
      | %<ID>
      | %<Vbase>V
      | %<VLF>pu
      | %<angleLF>deg.
      | %<Name>
  bus495 : powerlib/Measurements/Load Flow Bus  LConnTagsString=a  ID=bus495  Vbase=220000  Vref=1  Vangle=0  VLF=1  angleLF=0
      settings: AttributesFormatString=|
      | %<ID>
      | %<Vbase>V
      | %<VLF>pu
      | %<angleLF>deg.
      | %<Name>
  bus496 : powerlib/Measurements/Load Flow Bus  LConnTagsString=a  ID=bus496  Vbase=220000  Vref=1  Vangle=0  VLF=1  angleLF=0
      settings: AttributesFormatString=|
      | %<ID>
      | %<Vbase>V
      | %<VLF>pu
      | %<angleLF>deg.
      | %<Name>
  bus497 : powerlib/Measurements/Load Flow Bus  LConnTagsString=a  ID=bus497  Vbase=220000  Vref=1  Vangle=0  VLF=1  angleLF=0
      settings: AttributesFormatString=|
      | %<ID>
      | %<Vbase>V
      | %<VLF>pu
      | %<angleLF>deg.
      | %<Name>
  bus498 : powerlib/Measurements/Load Flow Bus  LConnTagsString=a  ID=bus498  Vbase=220000  Vref=1  Vangle=0  VLF=1  angleLF=0
      settings: AttributesFormatString=|
      | %<ID>
      | %<Vbase>V
      | %<VLF>pu
      | %<angleLF>deg.
      | %<Name>
  bus499 : powerlib/Measurements/Load Flow Bus  LConnTagsString=a  ID=bus499  Vbase=220000  Vref=1  Vangle=0  VLF=1  angleLF=0
      settings: AttributesFormatString=|
      | %<ID>
      | %<Vbase>V
      | %<VLF>pu
      | %<angleLF>deg.
      | %<Name>
  bus5 : powerlib/Measurements/Load Flow Bus  LConnTagsString=a  ID=bus5  Vbase=110000  Vref=1  Vangle=0  VLF=1  angleLF=0
      settings: AttributesFormatString=|
      | %<ID>
      | %<Vbase>V
      | %<VLF>pu
      | %<angleLF>deg.
      | %<Name>
  bus50 : powerlib/Measurements/Load Flow Bus  LConnTagsString=a  ID=bus50  Vbase=220000  Vref=1  Vangle=0  VLF=1  angleLF=0
      settings: AttributesFormatString=|
      | %<ID>
      | %<Vbase>V
      | %<VLF>pu
      | %<angleLF>deg.
      | %<Name>
  bus500 : powerlib/Measurements/Load Flow Bus  LConnTagsString=a  ID=bus500  Vbase=220000  Vref=1  Vangle=0  VLF=1  angleLF=0
      settings: AttributesFormatString=|
      | %<ID>
      | %<Vbase>V
      | %<VLF>pu
      | %<angleLF>deg.
      | %<Name>
  bus501 : powerlib/Measurements/Load Flow Bus  LConnTagsString=a  ID=bus501  Vbase=220000  Vref=1  Vangle=0  VLF=1  angleLF=0
      settings: AttributesFormatString=|
      | %<ID>
      | %<Vbase>V
      | %<VLF>pu
      | %<angleLF>deg.
      | %<Name>
  bus502 : powerlib/Measurements/Load Flow Bus  LConnTagsString=a  ID=bus502  Vbase=220000  Vref=1  Vangle=0  VLF=1  angleLF=0
      settings: AttributesFormatString=|
      | %<ID>
      | %<Vbase>V
      | %<VLF>pu
      | %<angleLF>deg.
      | %<Name>
  bus503 : powerlib/Measurements/Load Flow Bus  LConnTagsString=a  ID=bus503  Vbase=220000  Vref=1  Vangle=0  VLF=1  angleLF=0
      settings: AttributesFormatString=|
      | %<ID>
      | %<Vbase>V
      | %<VLF>pu
      | %<angleLF>deg.
      | %<Name>
  bus504 : powerlib/Measurements/Load Flow Bus  LConnTagsString=a  ID=bus504  Vbase=220000  Vref=1  Vangle=0  VLF=1  angleLF=0
      settings: AttributesFormatString=|
      | %<ID>
      | %<Vbase>V
      | %<VLF>pu
      | %<angleLF>deg.
      | %<Name>
  bus505 : powerlib/Measurements/Load Flow Bus  LConnTagsString=a  ID=bus505  Vbase=220000  Vref=1  Vangle=0  VLF=1  angleLF=0
      settings: AttributesFormatString=|
      | %<ID>
      | %<Vbase>V
      | %<VLF>pu
      | %<angleLF>deg.
      | %<Name>
  bus506 : powerlib/Measurements/Load Flow Bus  LConnTagsString=a  ID=bus506  Vbase=500000  Vref=1  Vangle=0  VLF=1  angleLF=0
      settings: AttributesFormatString=|
      | %<ID>
      | %<Vbase>V
      | %<VLF>pu
      | %<angleLF>deg.
      | %<Name>
  bus507 : powerlib/Measurements/Load Flow Bus  LConnTagsString=a  ID=bus507  Vbase=500000  Vref=1  Vangle=0  VLF=1  angleLF=0
      settings: AttributesFormatString=|
      | %<ID>
      | %<Vbase>V
      | %<VLF>pu
      | %<angleLF>deg.
      | %<Name>
  bus508 : powerlib/Measurements/Load Flow Bus  LConnTagsString=a  ID=bus508  Vbase=500000  Vref=1  Vangle=0  VLF=1  angleLF=0
      settings: AttributesFormatString=|
      | %<ID>
      | %<Vbase>V
      | %<VLF>pu
      | %<angleLF>deg.
      | %<Name>
  bus509 : powerlib/Measurements/Load Flow Bus  LConnTagsString=a  ID=bus509  Vbase=500000  Vref=1  Vangle=0  VLF=1  angleLF=0
      settings: AttributesFormatString=|
      | %<ID>
      | %<Vbase>V
      | %<VLF>pu
      | %<angleLF>deg.
      | %<Name>
  bus51 : powerlib/Measurements/Load Flow Bus  LConnTagsString=a  ID=bus51  Vbase=220000  Vref=1  Vangle=0  VLF=1  angleLF=0
      settings: AttributesFormatString=|
      | %<ID>
      | %<Vbase>V
      | %<VLF>pu
      | %<angleLF>deg.
      | %<Name>
  bus510 : powerlib/Measurements/Load Flow Bus  LConnTagsString=a  ID=bus510  Vbase=500000  Vref=1  Vangle=0  VLF=1  angleLF=0
      settings: AttributesFormatString=|
      | %<ID>
      | %<Vbase>V
      | %<VLF>pu
      | %<angleLF>deg.
      | %<Name>
  bus511 : powerlib/Measurements/Load Flow Bus  LConnTagsString=a  ID=bus511  Vbase=500000  Vref=1  Vangle=0  VLF=1  angleLF=0
      settings: AttributesFormatString=|
      | %<ID>
      | %<Vbase>V
      | %<VLF>pu
      | %<angleLF>deg.
      | %<Name>
  bus512 : powerlib/Measurements/Load Flow Bus  LConnTagsString=a  ID=bus512  Vbase=500000  Vref=1  Vangle=0  VLF=1  angleLF=0
      settings: AttributesFormatString=|
      | %<ID>
      | %<Vbase>V
      | %<VLF>pu
      | %<angleLF>deg.
      | %<Name>
  bus513 : powerlib/Measurements/Load Flow Bus  LConnTagsString=a  ID=bus513  Vbase=500000  Vref=1  Vangle=0  VLF=1  angleLF=0
      settings: AttributesFormatString=|
      | %<ID>
      | %<Vbase>V
      | %<VLF>pu
      | %<angleLF>deg.
      | %<Name>
  bus514 : powerlib/Measurements/Load Flow Bus  LConnTagsString=a  ID=bus514  Vbase=500000  Vref=1  Vangle=0  VLF=1  angleLF=0
      settings: AttributesFormatString=|
      | %<ID>
      | %<Vbase>V
      | %<VLF>pu
      | %<angleLF>deg.
      | %<Name>
  bus515 : powerlib/Measurements/Load Flow Bus  LConnTagsString=a  ID=bus515  Vbase=500000  Vref=1  Vangle=0  VLF=1  angleLF=0
      settings: AttributesFormatString=|
      | %<ID>
      | %<Vbase>V
      | %<VLF>pu
      | %<angleLF>deg.
      | %<Name>
  bus516 : powerlib/Measurements/Load Flow Bus  LConnTagsString=a  ID=bus516  Vbase=500000  Vref=1  Vangle=0  VLF=1  angleLF=0
      settings: AttributesFormatString=|
      | %<ID>
      | %<Vbase>V
      | %<VLF>pu
      | %<angleLF>deg.
      | %<Name>
  bus517 : powerlib/Measurements/Load Flow Bus  LConnTagsString=a  ID=bus517  Vbase=500000  Vref=1  Vangle=0  VLF=1  angleLF=0
      settings: AttributesFormatString=|
      | %<ID>
      | %<Vbase>V
      | %<VLF>pu
      | %<angleLF>deg.
      | %<Name>
  bus518 : powerlib/Measurements/Load Flow Bus  LConnTagsString=a  ID=bus518  Vbase=500000  Vref=1  Vangle=0  VLF=1  angleLF=0
      settings: AttributesFormatString=|
      | %<ID>
      | %<Vbase>V
      | %<VLF>pu
      | %<angleLF>deg.
      | %<Name>
  bus519 : powerlib/Measurements/Load Flow Bus  LConnTagsString=a  ID=bus519  Vbase=500000  Vref=1  Vangle=0  VLF=1  angleLF=0
      settings: AttributesFormatString=|
      | %<ID>
      | %<Vbase>V
      | %<VLF>pu
      | %<angleLF>deg.
      | %<Name>
  bus52 : powerlib/Measurements/Load Flow Bus  LConnTagsString=a  ID=bus52  Vbase=220000  Vref=1  Vangle=0  VLF=1  angleLF=0
      settings: AttributesFormatString=|
      | %<ID>
      | %<Vbase>V
      | %<VLF>pu
      | %<angleLF>deg.
      | %<Name>
  bus520 : powerlib/Measurements/Load Flow Bus  LConnTagsString=a  ID=bus520  Vbase=500000  Vref=1  Vangle=0  VLF=1  angleLF=0
      settings: AttributesFormatString=|
      | %<ID>
      | %<Vbase>V
      | %<VLF>pu
      | %<angleLF>deg.
      | %<Name>
  bus521 : powerlib/Measurements/Load Flow Bus  LConnTagsString=a  ID=bus521  Vbase=500000  Vref=1  Vangle=0  VLF=1  angleLF=0
      settings: AttributesFormatString=|
      | %<ID>
      | %<Vbase>V
      | %<VLF>pu
      | %<angleLF>deg.
      | %<Name>
  bus522 : powerlib/Measurements/Load Flow Bus  LConnTagsString=a  ID=bus522  Vbase=500000  Vref=1  Vangle=0  VLF=1  angleLF=0
      settings: AttributesFormatString=|
      | %<ID>
      | %<Vbase>V
      | %<VLF>pu
      | %<angleLF>deg.
      | %<Name>
  bus523 : powerlib/Measurements/Load Flow Bus  LConnTagsString=a  ID=bus523  Vbase=500000  Vref=1  Vangle=0  VLF=1  angleLF=0
      settings: AttributesFormatString=|
      | %<ID>
      | %<Vbase>V
      | %<VLF>pu
      | %<angleLF>deg.
      | %<Name>
  bus524 : powerlib/Measurements/Load Flow Bus  LConnTagsString=a  ID=bus524  Vbase=500000  Vref=1  Vangle=0  VLF=1  angleLF=0
      settings: AttributesFormatString=|
      | %<ID>
      | %<Vbase>V
      | %<VLF>pu
      | %<angleLF>deg.
      | %<Name>
  bus525 : powerlib/Measurements/Load Flow Bus  LConnTagsString=a  ID=bus525  Vbase=500000  Vref=1  Vangle=0  VLF=1  angleLF=0
      settings: AttributesFormatString=|
      | %<ID>
      | %<Vbase>V
      | %<VLF>pu
      | %<angleLF>deg.
      | %<Name>
  bus526 : powerlib/Measurements/Load Flow Bus  LConnTagsString=a  ID=bus526  Vbase=500000  Vref=1  Vangle=0  VLF=1  angleLF=0
      settings: AttributesFormatString=|
      | %<ID>
      | %<Vbase>V
      | %<VLF>pu
      | %<angleLF>deg.
      | %<Name>
  bus527 : powerlib/Measurements/Load Flow Bus  LConnTagsString=a  ID=bus527  Vbase=500000  Vref=1  Vangle=0  VLF=1  angleLF=0
      settings: AttributesFormatString=|
      | %<ID>
      | %<Vbase>V
      | %<VLF>pu
      | %<angleLF>deg.
      | %<Name>
  bus528 : powerlib/Measurements/Load Flow Bus  LConnTagsString=a  ID=bus528  Vbase=500000  Vref=1  Vangle=0  VLF=1  angleLF=0
      settings: AttributesFormatString=|
      | %<ID>
      | %<Vbase>V
      | %<VLF>pu
      | %<angleLF>deg.
      | %<Name>
  bus529 : powerlib/Measurements/Load Flow Bus  LConnTagsString=a  ID=bus529  Vbase=500000  Vref=1  Vangle=0  VLF=1  angleLF=0
      settings: AttributesFormatString=|
      | %<ID>
      | %<Vbase>V
      | %<VLF>pu
      | %<angleLF>deg.
      | %<Name>
  bus53 : powerlib/Measurements/Load Flow Bus  LConnTagsString=a  ID=bus53  Vbase=220000  Vref=1  Vangle=0  VLF=1  angleLF=0
      settings: AttributesFormatString=|
      | %<ID>
      | %<Vbase>V
      | %<VLF>pu
      | %<angleLF>deg.
      | %<Name>
  bus530 : powerlib/Measurements/Load Flow Bus  LConnTagsString=a  ID=bus530  Vbase=500000  Vref=1  Vangle=0  VLF=1  angleLF=0
      settings: AttributesFormatString=|
      | %<ID>
      | %<Vbase>V
      | %<VLF>pu
      | %<angleLF>deg.
      | %<Name>
  bus531 : powerlib/Measurements/Load Flow Bus  LConnTagsString=a  ID=bus531  Vbase=500000  Vref=1  Vangle=0  VLF=1  angleLF=0
      settings: AttributesFormatString=|
      | %<ID>
      | %<Vbase>V
      | %<VLF>pu
      | %<angleLF>deg.
      | %<Name>
  bus532 : powerlib/Measurements/Load Flow Bus  LConnTagsString=a  ID=bus532  Vbase=500000  Vref=1  Vangle=0  VLF=1  angleLF=0
      settings: AttributesFormatString=|
      | %<ID>
      | %<Vbase>V
      | %<VLF>pu
      | %<angleLF>deg.
      | %<Name>
  bus533 : powerlib/Measurements/Load Flow Bus  LConnTagsString=a  ID=bus533  Vbase=500000  Vref=1  Vangle=0  VLF=1  angleLF=0
      settings: AttributesFormatString=|
      | %<ID>
      | %<Vbase>V
      | %<VLF>pu
      | %<angleLF>deg.
      | %<Name>
  bus534 : powerlib/Measurements/Load Flow Bus  LConnTagsString=a  ID=bus534  Vbase=500000  Vref=1  Vangle=0  VLF=1  angleLF=0
      settings: AttributesFormatString=|
      | %<ID>
      | %<Vbase>V
      | %<VLF>pu
      | %<angleLF>deg.
      | %<Name>
  bus535 : powerlib/Measurements/Load Flow Bus  LConnTagsString=a  ID=bus535  Vbase=500000  Vref=1  Vangle=0  VLF=1  angleLF=0
      settings: AttributesFormatString=|
      | %<ID>
      | %<Vbase>V
      | %<VLF>pu
      | %<angleLF>deg.
      | %<Name>
  bus536 : powerlib/Measurements/Load Flow Bus  LConnTagsString=a  ID=bus536  Vbase=500000  Vref=1  Vangle=0  VLF=1  angleLF=0
      settings: AttributesFormatString=|
      | %<ID>
      | %<Vbase>V
      | %<VLF>pu
      | %<angleLF>deg.
      | %<Name>
  bus537 : powerlib/Measurements/Load Flow Bus  LConnTagsString=a  ID=bus537  Vbase=500000  Vref=1  Vangle=0  VLF=1  angleLF=0
      settings: AttributesFormatString=|
      | %<ID>
      | %<Vbase>V
      | %<VLF>pu
      | %<angleLF>deg.
      | %<Name>
  bus538 : powerlib/Measurements/Load Flow Bus  LConnTagsString=a  ID=bus538  Vbase=500000  Vref=1  Vangle=0  VLF=1  angleLF=0
      settings: AttributesFormatString=|
      | %<ID>
      | %<Vbase>V
      | %<VLF>pu
      | %<angleLF>deg.
      | %<Name>
  bus539 : powerlib/Measurements/Load Flow Bus  LConnTagsString=a  ID=bus539  Vbase=500000  Vref=1  Vangle=0  VLF=1  angleLF=0
      settings: AttributesFormatString=|
      | %<ID>
      | %<Vbase>V
      | %<VLF>pu
      | %<angleLF>deg.
      | %<Name>
  bus54 : powerlib/Measurements/Load Flow Bus  LConnTagsString=a  ID=bus54  Vbase=220000  Vref=1  Vangle=0  VLF=1  angleLF=0
      settings: AttributesFormatString=|
      | %<ID>
      | %<Vbase>V
      | %<VLF>pu
      | %<angleLF>deg.
      | %<Name>
  bus540 : powerlib/Measurements/Load Flow Bus  LConnTagsString=a  ID=bus540  Vbase=500000  Vref=1  Vangle=0  VLF=1  angleLF=0
      settings: AttributesFormatString=|
      | %<ID>
      | %<Vbase>V
      | %<VLF>pu
      | %<angleLF>deg.
      | %<Name>
  bus541 : powerlib/Measurements/Load Flow Bus  LConnTagsString=a  ID=bus541  Vbase=500000  Vref=1  Vangle=0  VLF=1  angleLF=0
      settings: AttributesFormatString=|
      | %<ID>
      | %<Vbase>V
      | %<VLF>pu
      | %<angleLF>deg.
      | %<Name>
  bus542 : powerlib/Measurements/Load Flow Bus  LConnTagsString=a  ID=bus542  Vbase=500000  Vref=1  Vangle=0  VLF=1  angleLF=0
      settings: AttributesFormatString=|
      | %<ID>
      | %<Vbase>V
      | %<VLF>pu
      | %<angleLF>deg.
      | %<Name>
  bus543 : powerlib/Measurements/Load Flow Bus  LConnTagsString=a  ID=bus543  Vbase=500000  Vref=1  Vangle=0  VLF=1  angleLF=0
      settings: AttributesFormatString=|
      | %<ID>
      | %<Vbase>V
      | %<VLF>pu
      | %<angleLF>deg.
      | %<Name>
  bus544 : powerlib/Measurements/Load Flow Bus  LConnTagsString=a  ID=bus544  Vbase=500000  Vref=1  Vangle=0  VLF=1  angleLF=0
      settings: AttributesFormatString=|
      | %<ID>
      | %<Vbase>V
      | %<VLF>pu
      | %<angleLF>deg.
      | %<Name>
  bus545 : powerlib/Measurements/Load Flow Bus  LConnTagsString=a  ID=bus545  Vbase=500000  Vref=1  Vangle=0  VLF=1  angleLF=0
      settings: AttributesFormatString=|
      | %<ID>
      | %<Vbase>V
      | %<VLF>pu
      | %<angleLF>deg.
      | %<Name>
  bus546 : powerlib/Measurements/Load Flow Bus  LConnTagsString=a  ID=bus546  Vbase=500000  Vref=1  Vangle=0  VLF=1  angleLF=0
      settings: AttributesFormatString=|
      | %<ID>
      | %<Vbase>V
      | %<VLF>pu
      | %<angleLF>deg.
      | %<Name>
  bus547 : powerlib/Measurements/Load Flow Bus  LConnTagsString=a  ID=bus547  Vbase=500000  Vref=1  Vangle=0  VLF=1  angleLF=0
      settings: AttributesFormatString=|
      | %<ID>
      | %<Vbase>V
      | %<VLF>pu
      | %<angleLF>deg.
      | %<Name>
  bus548 : powerlib/Measurements/Load Flow Bus  LConnTagsString=a  ID=bus548  Vbase=500000  Vref=1  Vangle=0  VLF=1  angleLF=0
      settings: AttributesFormatString=|
      | %<ID>
      | %<Vbase>V
      | %<VLF>pu
      | %<angleLF>deg.
      | %<Name>
  bus549 : powerlib/Measurements/Load Flow Bus  LConnTagsString=a  ID=bus549  Vbase=500000  Vref=1  Vangle=0  VLF=1  angleLF=0
      settings: AttributesFormatString=|
      | %<ID>
      | %<Vbase>V
      | %<VLF>pu
      | %<angleLF>deg.
      | %<Name>
  bus55 : powerlib/Measurements/Load Flow Bus  LConnTagsString=a  ID=bus55  Vbase=220000  Vref=1  Vangle=0  VLF=1  angleLF=0
      settings: AttributesFormatString=|
      | %<ID>
      | %<Vbase>V
      | %<VLF>pu
      | %<angleLF>deg.
      | %<Name>
  bus550 : powerlib/Measurements/Load Flow Bus  LConnTagsString=a  ID=bus550  Vbase=500000  Vref=1  Vangle=0  VLF=1  angleLF=0
      settings: AttributesFormatString=|
      | %<ID>
      | %<Vbase>V
      | %<VLF>pu
      | %<angleLF>deg.
      | %<Name>
  bus551 : powerlib/Measurements/Load Flow Bus  LConnTagsString=a  ID=bus551  Vbase=500000  Vref=1  Vangle=0  VLF=1  angleLF=0
      settings: AttributesFormatString=|
      | %<ID>
      | %<Vbase>V
      | %<VLF>pu
      | %<angleLF>deg.
      | %<Name>
  bus552 : powerlib/Measurements/Load Flow Bus  LConnTagsString=a  ID=bus552  Vbase=500000  Vref=1  Vangle=0  VLF=1  angleLF=0
      settings: AttributesFormatString=|
      | %<ID>
      | %<Vbase>V
      | %<VLF>pu
      | %<angleLF>deg.
      | %<Name>
  bus553 : powerlib/Measurements/Load Flow Bus  LConnTagsString=a  ID=bus553  Vbase=500000  Vref=1  Vangle=0  VLF=1  angleLF=0
      settings: AttributesFormatString=|
      | %<ID>
      | %<Vbase>V
      | %<VLF>pu
      | %<angleLF>deg.
      | %<Name>
  bus554 : powerlib/Measurements/Load Flow Bus  LConnTagsString=a  ID=bus554  Vbase=500000  Vref=1  Vangle=0  VLF=1  angleLF=0
      settings: AttributesFormatString=|
      | %<ID>
      | %<Vbase>V
      | %<VLF>pu
      | %<angleLF>deg.
      | %<Name>
  bus555 : powerlib/Measurements/Load Flow Bus  LConnTagsString=a  ID=bus555  Vbase=500000  Vref=1  Vangle=0  VLF=1  angleLF=0
      settings: AttributesFormatString=|
      | %<ID>
      | %<Vbase>V
      | %<VLF>pu
      | %<angleLF>deg.
      | %<Name>
  bus556 : powerlib/Measurements/Load Flow Bus  LConnTagsString=a  ID=bus556  Vbase=500000  Vref=1  Vangle=0  VLF=1  angleLF=0
      settings: AttributesFormatString=|
      | %<ID>
      | %<Vbase>V
      | %<VLF>pu
      | %<angleLF>deg.
      | %<Name>
  bus557 : powerlib/Measurements/Load Flow Bus  LConnTagsString=a  ID=bus557  Vbase=500000  Vref=1  Vangle=0  VLF=1  angleLF=0
      settings: AttributesFormatString=|
      | %<ID>
      | %<Vbase>V
      | %<VLF>pu
      | %<angleLF>deg.
      | %<Name>
  bus558 : powerlib/Measurements/Load Flow Bus  LConnTagsString=a  ID=bus558  Vbase=500000  Vref=1  Vangle=0  VLF=1  angleLF=0
      settings: AttributesFormatString=|
      | %<ID>
      | %<Vbase>V
      | %<VLF>pu
      | %<angleLF>deg.
      | %<Name>
  bus559 : powerlib/Measurements/Load Flow Bus  LConnTagsString=a  ID=bus559  Vbase=500000  Vref=1  Vangle=0  VLF=1  angleLF=0
      settings: AttributesFormatString=|
      | %<ID>
      | %<Vbase>V
      | %<VLF>pu
      | %<angleLF>deg.
      | %<Name>
  bus56 : powerlib/Measurements/Load Flow Bus  LConnTagsString=a  ID=bus56  Vbase=220000  Vref=1  Vangle=0  VLF=1  angleLF=0
      settings: AttributesFormatString=|
      | %<ID>
      | %<Vbase>V
      | %<VLF>pu
      | %<angleLF>deg.
      | %<Name>
  bus560 : powerlib/Measurements/Load Flow Bus  LConnTagsString=a  ID=bus560  Vbase=500000  Vref=1  Vangle=0  VLF=1  angleLF=0
      settings: AttributesFormatString=|
      | %<ID>
      | %<Vbase>V
      | %<VLF>pu
      | %<angleLF>deg.
      | %<Name>
  bus561 : powerlib/Measurements/Load Flow Bus  LConnTagsString=a  ID=bus561  Vbase=500000  Vref=1  Vangle=0  VLF=1  angleLF=0
      settings: AttributesFormatString=|
      | %<ID>
      | %<Vbase>V
      | %<VLF>pu
      | %<angleLF>deg.
      | %<Name>
  bus562 : powerlib/Measurements/Load Flow Bus  LConnTagsString=a  ID=bus562  Vbase=500000  Vref=1  Vangle=0  VLF=1  angleLF=0
      settings: AttributesFormatString=|
      | %<ID>
      | %<Vbase>V
      | %<VLF>pu
      | %<angleLF>deg.
      | %<Name>
  bus563 : powerlib/Measurements/Load Flow Bus  LConnTagsString=a  ID=bus563  Vbase=500000  Vref=1  Vangle=0  VLF=1  angleLF=0
      settings: AttributesFormatString=|
      | %<ID>
      | %<Vbase>V
      | %<VLF>pu
      | %<angleLF>deg.
      | %<Name>
  bus564 : powerlib/Measurements/Load Flow Bus  LConnTagsString=a  ID=bus564  Vbase=500000  Vref=1  Vangle=0  VLF=1  angleLF=0
      settings: AttributesFormatString=|
      | %<ID>
      | %<Vbase>V
      | %<VLF>pu
      | %<angleLF>deg.
      | %<Name>
  bus565 : powerlib/Measurements/Load Flow Bus  LConnTagsString=a  ID=bus565  Vbase=500000  Vref=1  Vangle=0  VLF=1  angleLF=0
      settings: AttributesFormatString=|
      | %<ID>
      | %<Vbase>V
      | %<VLF>pu
      | %<angleLF>deg.
      | %<Name>
  bus566 : powerlib/Measurements/Load Flow Bus  LConnTagsString=a  ID=bus566  Vbase=500000  Vref=1  Vangle=0  VLF=1  angleLF=0
      settings: AttributesFormatString=|
      | %<ID>
      | %<Vbase>V
      | %<VLF>pu
      | %<angleLF>deg.
      | %<Name>
  bus567 : powerlib/Measurements/Load Flow Bus  LConnTagsString=a  ID=bus567  Vbase=500000  Vref=1  Vangle=0  VLF=1  angleLF=0
      settings: AttributesFormatString=|
      | %<ID>
      | %<Vbase>V
      | %<VLF>pu
      | %<angleLF>deg.
      | %<Name>
  bus568 : powerlib/Measurements/Load Flow Bus  LConnTagsString=a  ID=bus568  Vbase=500000  Vref=1  Vangle=0  VLF=1  angleLF=0
      settings: AttributesFormatString=|
      | %<ID>
      | %<Vbase>V
      | %<VLF>pu
      | %<angleLF>deg.
      | %<Name>
  bus569 : powerlib/Measurements/Load Flow Bus  LConnTagsString=a  ID=bus569  Vbase=500000  Vref=1  Vangle=0  VLF=1  angleLF=0
      settings: AttributesFormatString=|
      | %<ID>
      | %<Vbase>V
      | %<VLF>pu
      | %<angleLF>deg.
      | %<Name>
  bus57 : powerlib/Measurements/Load Flow Bus  LConnTagsString=a  ID=bus57  Vbase=220000  Vref=1  Vangle=0  VLF=1  angleLF=0
      settings: AttributesFormatString=|
      | %<ID>
      | %<Vbase>V
      | %<VLF>pu
      | %<angleLF>deg.
      | %<Name>
  bus570 : powerlib/Measurements/Load Flow Bus  LConnTagsString=a  ID=bus570  Vbase=500000  Vref=1  Vangle=0  VLF=1  angleLF=0
      settings: AttributesFormatString=|
      | %<ID>
      | %<Vbase>V
      | %<VLF>pu
      | %<angleLF>deg.
      | %<Name>
  bus571 : powerlib/Measurements/Load Flow Bus  LConnTagsString=a  ID=bus571  Vbase=500000  Vref=1  Vangle=0  VLF=1  angleLF=0
      settings: AttributesFormatString=|
      | %<ID>
      | %<Vbase>V
      | %<VLF>pu
      | %<angleLF>deg.
      | %<Name>
  bus572 : powerlib/Measurements/Load Flow Bus  LConnTagsString=a  ID=bus572  Vbase=500000  Vref=1  Vangle=0  VLF=1  angleLF=0
      settings: AttributesFormatString=|
      | %<ID>
      | %<Vbase>V
      | %<VLF>pu
      | %<angleLF>deg.
      | %<Name>
  bus573 : powerlib/Measurements/Load Flow Bus  LConnTagsString=a  ID=bus573  Vbase=500000  Vref=1  Vangle=0  VLF=1  angleLF=0
      settings: AttributesFormatString=|
      | %<ID>
      | %<Vbase>V
      | %<VLF>pu
      | %<angleLF>deg.
      | %<Name>
  bus574 : powerlib/Measurements/Load Flow Bus  LConnTagsString=a  ID=bus574  Vbase=500000  Vref=1  Vangle=0  VLF=1  angleLF=0
      settings: AttributesFormatString=|
      | %<ID>
      | %<Vbase>V
      | %<VLF>pu
      | %<angleLF>deg.
      | %<Name>
  bus575 : powerlib/Measurements/Load Flow Bus  LConnTagsString=a  ID=bus575  Vbase=500000  Vref=1  Vangle=0  VLF=1  angleLF=0
      settings: AttributesFormatString=|
      | %<ID>
      | %<Vbase>V
      | %<VLF>pu
      | %<angleLF>deg.
      | %<Name>
  bus576 : powerlib/Measurements/Load Flow Bus  LConnTagsString=a  ID=bus576  Vbase=500000  Vref=1  Vangle=0  VLF=1  angleLF=0
      settings: AttributesFormatString=|
      | %<ID>
      | %<Vbase>V
      | %<VLF>pu
      | %<angleLF>deg.
      | %<Name>
  bus577 : powerlib/Measurements/Load Flow Bus  LConnTagsString=a  ID=bus577  Vbase=500000  Vref=1  Vangle=0  VLF=1  angleLF=0
      settings: AttributesFormatString=|
      | %<ID>
      | %<Vbase>V
      | %<VLF>pu
      | %<angleLF>deg.
      | %<Name>
  bus578 : powerlib/Measurements/Load Flow Bus  LConnTagsString=a  ID=bus578  Vbase=500000  Vref=1  Vangle=0  VLF=1  angleLF=0
      settings: AttributesFormatString=|
      | %<ID>
      | %<Vbase>V
      | %<VLF>pu
      | %<angleLF>deg.
      | %<Name>
  bus579 : powerlib/Measurements/Load Flow Bus  LConnTagsString=a  ID=bus579  Vbase=500000  Vref=1  Vangle=0  VLF=1  angleLF=0
      settings: AttributesFormatString=|
      | %<ID>
      | %<Vbase>V
      | %<VLF>pu
      | %<angleLF>deg.
      | %<Name>
  bus58 : powerlib/Measurements/Load Flow Bus  LConnTagsString=a  ID=bus58  Vbase=220000  Vref=1  Vangle=0  VLF=1  angleLF=0
      settings: AttributesFormatString=|
      | %<ID>
      | %<Vbase>V
      | %<VLF>pu
      | %<angleLF>deg.
      | %<Name>
  bus580 : powerlib/Measurements/Load Flow Bus  LConnTagsString=a  ID=bus580  Vbase=500000  Vref=1  Vangle=0  VLF=1  angleLF=0
      settings: AttributesFormatString=|
      | %<ID>
      | %<Vbase>V
      | %<VLF>pu
      | %<angleLF>deg.
      | %<Name>
  bus581 : powerlib/Measurements/Load Flow Bus  LConnTagsString=a  ID=bus581  Vbase=500000  Vref=1  Vangle=0  VLF=1  angleLF=0
      settings: AttributesFormatString=|
      | %<ID>
      | %<Vbase>V
      | %<VLF>pu
      | %<angleLF>deg.
      | %<Name>
  bus582 : powerlib/Measurements/Load Flow Bus  LConnTagsString=a  ID=bus582  Vbase=500000  Vref=1  Vangle=0  VLF=1  angleLF=0
      settings: AttributesFormatString=|
      | %<ID>
      | %<Vbase>V
      | %<VLF>pu
      | %<angleLF>deg.
      | %<Name>
  bus583 : powerlib/Measurements/Load Flow Bus  LConnTagsString=a  ID=bus583  Vbase=500000  Vref=1  Vangle=0  VLF=1  angleLF=0
      settings: AttributesFormatString=|
      | %<ID>
      | %<Vbase>V
      | %<VLF>pu
      | %<angleLF>deg.
      | %<Name>
  bus59 : powerlib/Measurements/Load Flow Bus  LConnTagsString=a  ID=bus59  Vbase=220000  Vref=1  Vangle=0  VLF=1  angleLF=0
      settings: AttributesFormatString=|
      | %<ID>
      | %<Vbase>V
      | %<VLF>pu
      | %<angleLF>deg.
      | %<Name>
  bus6 : powerlib/Measurements/Load Flow Bus  LConnTagsString=a  ID=bus6  Vbase=110000  Vref=1  Vangle=0  VLF=1  angleLF=0
      settings: AttributesFormatString=|
      | %<ID>
      | %<Vbase>V
      | %<VLF>pu
      | %<angleLF>deg.
      | %<Name>
  bus60 : powerlib/Measurements/Load Flow Bus  LConnTagsString=a  ID=bus60  Vbase=220000  Vref=1  Vangle=0  VLF=1  angleLF=0
      settings: AttributesFormatString=|
      | %<ID>
      | %<Vbase>V
      | %<VLF>pu
      | %<angleLF>deg.
      | %<Name>
  bus61 : powerlib/Measurements/Load Flow Bus  LConnTagsString=a  ID=bus61  Vbase=220000  Vref=1  Vangle=0  VLF=1  angleLF=0
      settings: AttributesFormatString=|
      | %<ID>
      | %<Vbase>V
      | %<VLF>pu
      | %<angleLF>deg.
      | %<Name>
  bus62 : powerlib/Measurements/Load Flow Bus  LConnTagsString=a  ID=bus62  Vbase=220000  Vref=1  Vangle=0  VLF=1  angleLF=0
      settings: AttributesFormatString=|
      | %<ID>
      | %<Vbase>V
      | %<VLF>pu
      | %<angleLF>deg.
      | %<Name>
  bus63 : powerlib/Measurements/Load Flow Bus  LConnTagsString=a  ID=bus63  Vbase=220000  Vref=1  Vangle=0  VLF=1  angleLF=0
      settings: AttributesFormatString=|
      | %<ID>
      | %<Vbase>V
      | %<VLF>pu
      | %<angleLF>deg.
      | %<Name>
  bus64 : powerlib/Measurements/Load Flow Bus  LConnTagsString=a  ID=bus64  Vbase=220000  Vref=1  Vangle=0  VLF=1  angleLF=0
      settings: AttributesFormatString=|
      | %<ID>
      | %<Vbase>V
      | %<VLF>pu
      | %<angleLF>deg.
      | %<Name>
  bus65 : powerlib/Measurements/Load Flow Bus  LConnTagsString=a  ID=bus65  Vbase=220000  Vref=1  Vangle=0  VLF=1  angleLF=0
      settings: AttributesFormatString=|
      | %<ID>
      | %<Vbase>V
      | %<VLF>pu
      | %<angleLF>deg.
      | %<Name>
  bus66 : powerlib/Measurements/Load Flow Bus  LConnTagsString=a  ID=bus66  Vbase=220000  Vref=1  Vangle=0  VLF=1  angleLF=0
      settings: AttributesFormatString=|
      | %<ID>
      | %<Vbase>V
      | %<VLF>pu
      | %<angleLF>deg.
      | %<Name>
  bus67 : powerlib/Measurements/Load Flow Bus  LConnTagsString=a  ID=bus67  Vbase=220000  Vref=1  Vangle=0  VLF=1  angleLF=0
      settings: AttributesFormatString=|
      | %<ID>
      | %<Vbase>V
      | %<VLF>pu
      | %<angleLF>deg.
      | %<Name>
  bus68 : powerlib/Measurements/Load Flow Bus  LConnTagsString=a  ID=bus68  Vbase=220000  Vref=1  Vangle=0  VLF=1  angleLF=0
      settings: AttributesFormatString=|
      | %<ID>
      | %<Vbase>V
      | %<VLF>pu
      | %<angleLF>deg.
      | %<Name>
  bus69 : powerlib/Measurements/Load Flow Bus  LConnTagsString=a  ID=bus69  Vbase=220000  Vref=1  Vangle=0  VLF=1  angleLF=0
      settings: AttributesFormatString=|
      | %<ID>
      | %<Vbase>V
      | %<VLF>pu
      | %<angleLF>deg.
      | %<Name>
  bus7 : powerlib/Measurements/Load Flow Bus  LConnTagsString=a  ID=bus7  Vbase=110000  Vref=1  Vangle=0  VLF=1  angleLF=0
      settings: AttributesFormatString=|
      | %<ID>
      | %<Vbase>V
      | %<VLF>pu
      | %<angleLF>deg.
      | %<Name>
  bus70 : powerlib/Measurements/Load Flow Bus  LConnTagsString=a  ID=bus70  Vbase=220000  Vref=1  Vangle=0  VLF=1  angleLF=0
      settings: AttributesFormatString=|
      | %<ID>
      | %<Vbase>V
      | %<VLF>pu
      | %<angleLF>deg.
      | %<Name>
  bus71 : powerlib/Measurements/Load Flow Bus  LConnTagsString=a  ID=bus71  Vbase=220000  Vref=1  Vangle=0  VLF=1  angleLF=0
      settings: AttributesFormatString=|
      | %<ID>
      | %<Vbase>V
      | %<VLF>pu
      | %<angleLF>deg.
      | %<Name>
  bus72 : powerlib/Measurements/Load Flow Bus  LConnTagsString=a  ID=bus72  Vbase=220000  Vref=1  Vangle=0  VLF=1  angleLF=0
      settings: AttributesFormatString=|
      | %<ID>
      | %<Vbase>V
      | %<VLF>pu
      | %<angleLF>deg.
      | %<Name>
  bus73 : powerlib/Measurements/Load Flow Bus  LConnTagsString=a  ID=bus73  Vbase=220000  Vref=1  Vangle=0  VLF=1  angleLF=0
      settings: AttributesFormatString=|
      | %<ID>
      | %<Vbase>V
      | %<VLF>pu
      | %<angleLF>deg.
      | %<Name>
  bus74 : powerlib/Measurements/Load Flow Bus  LConnTagsString=a  ID=bus74  Vbase=220000  Vref=1  Vangle=0  VLF=1  angleLF=0
      settings: AttributesFormatString=|
      | %<ID>
      | %<Vbase>V
      | %<VLF>pu
      | %<angleLF>deg.
      | %<Name>
  bus75 : powerlib/Measurements/Load Flow Bus  LConnTagsString=a  ID=bus75  Vbase=220000  Vref=1  Vangle=0  VLF=1  angleLF=0
      settings: AttributesFormatString=|
      | %<ID>
      | %<Vbase>V
      | %<VLF>pu
      | %<angleLF>deg.
      | %<Name>
  bus76 : powerlib/Measurements/Load Flow Bus  LConnTagsString=a  ID=bus76  Vbase=220000  Vref=1  Vangle=0  VLF=1  angleLF=0
      settings: AttributesFormatString=|
      | %<ID>
      | %<Vbase>V
      | %<VLF>pu
      | %<angleLF>deg.
      | %<Name>
  bus77 : powerlib/Measurements/Load Flow Bus  LConnTagsString=a  ID=bus77  Vbase=220000  Vref=1  Vangle=0  VLF=1  angleLF=0
      settings: AttributesFormatString=|
      | %<ID>
      | %<Vbase>V
      | %<VLF>pu
      | %<angleLF>deg.
      | %<Name>
  bus78 : powerlib/Measurements/Load Flow Bus  LConnTagsString=a  ID=bus78  Vbase=220000  Vref=1  Vangle=0  VLF=1  angleLF=0
      settings: AttributesFormatString=|
      | %<ID>
      | %<Vbase>V
      | %<VLF>pu
      | %<angleLF>deg.
      | %<Name>
  bus79 : powerlib/Measurements/Load Flow Bus  LConnTagsString=a  ID=bus79  Vbase=220000  Vref=1  Vangle=0  VLF=1  angleLF=0
      settings: AttributesFormatString=|
      | %<ID>
      | %<Vbase>V
      | %<VLF>pu
      | %<angleLF>deg.
      | %<Name>
  bus8 : powerlib/Measurements/Load Flow Bus  LConnTagsString=a  ID=bus8  Vbase=110000  Vref=1  Vangle=0  VLF=1  angleLF=0
      settings: AttributesFormatString=|
      | %<ID>
      | %<Vbase>V
      | %<VLF>pu
      | %<angleLF>deg.
      | %<Name>
  bus80 : powerlib/Measurements/Load Flow Bus  LConnTagsString=a  ID=bus80  Vbase=220000  Vref=1  Vangle=0  VLF=1  angleLF=0
      settings: AttributesFormatString=|
      | %<ID>
      | %<Vbase>V
      | %<VLF>pu
      | %<angleLF>deg.
      | %<Name>
  bus81 : powerlib/Measurements/Load Flow Bus  LConnTagsString=a  ID=bus81  Vbase=220000  Vref=1  Vangle=0  VLF=1  angleLF=0
      settings: AttributesFormatString=|
      | %<ID>
      | %<Vbase>V
      | %<VLF>pu
      | %<angleLF>deg.
      | %<Name>
  bus82 : powerlib/Measurements/Load Flow Bus  LConnTagsString=a  ID=bus82  Vbase=220000  Vref=1  Vangle=0  VLF=1  angleLF=0
      settings: AttributesFormatString=|
      | %<ID>
      | %<Vbase>V
      | %<VLF>pu
      | %<angleLF>deg.
      | %<Name>
  bus83 : powerlib/Measurements/Load Flow Bus  LConnTagsString=a  ID=bus83  Vbase=220000  Vref=1  Vangle=0  VLF=1  angleLF=0
      settings: AttributesFormatString=|
      | %<ID>
      | %<Vbase>V
      | %<VLF>pu
      | %<angleLF>deg.
      | %<Name>
  bus84 : powerlib/Measurements/Load Flow Bus  LConnTagsString=a  ID=bus84  Vbase=220000  Vref=1  Vangle=0  VLF=1  angleLF=0
      settings: AttributesFormatString=|
      | %<ID>
      | %<Vbase>V
      | %<VLF>pu
      | %<angleLF>deg.
      | %<Name>
  bus85 : powerlib/Measurements/Load Flow Bus  LConnTagsString=a  ID=bus85  Vbase=220000  Vref=1  Vangle=0  VLF=1  angleLF=0
      settings: AttributesFormatString=|
      | %<ID>
      | %<Vbase>V
      | %<VLF>pu
      | %<angleLF>deg.
      | %<Name>
  bus86 : powerlib/Measurements/Load Flow Bus  LConnTagsString=a  ID=bus86  Vbase=220000  Vref=1  Vangle=0  VLF=1  angleLF=0
      settings: AttributesFormatString=|
      | %<ID>
      | %<Vbase>V
      | %<VLF>pu
      | %<angleLF>deg.
      | %<Name>
  bus87 : powerlib/Measurements/Load Flow Bus  LConnTagsString=a  ID=bus87  Vbase=220000  Vref=1  Vangle=0  VLF=1  angleLF=0
      settings: AttributesFormatString=|
      | %<ID>
      | %<Vbase>V
      | %<VLF>pu
      | %<angleLF>deg.
      | %<Name>
  bus88 : powerlib/Measurements/Load Flow Bus  LConnTagsString=a  ID=bus88  Vbase=220000  Vref=1  Vangle=0  VLF=1  angleLF=0
      settings: AttributesFormatString=|
      | %<ID>
      | %<Vbase>V
      | %<VLF>pu
      | %<angleLF>deg.
      | %<Name>
  bus89 : powerlib/Measurements/Load Flow Bus  LConnTagsString=a  ID=bus89  Vbase=220000  Vref=1  Vangle=0  VLF=1  angleLF=0
      settings: AttributesFormatString=|
      | %<ID>
      | %<Vbase>V
      | %<VLF>pu
      | %<angleLF>deg.
      | %<Name>
  bus9 : powerlib/Measurements/Load Flow Bus  LConnTagsString=a  ID=bus9  Vbase=110000  Vref=1  Vangle=0  VLF=1  angleLF=0
      settings: AttributesFormatString=|
      | %<ID>
      | %<Vbase>V
      | %<VLF>pu
      | %<angleLF>deg.
      | %<Name>
  bus90 : powerlib/Measurements/Load Flow Bus  LConnTagsString=a  ID=bus90  Vbase=220000  Vref=1  Vangle=0  VLF=1  angleLF=0
      settings: AttributesFormatString=|
      | %<ID>
      | %<Vbase>V
      | %<VLF>pu
      | %<angleLF>deg.
      | %<Name>
  bus91 : powerlib/Measurements/Load Flow Bus  LConnTagsString=a  ID=bus91  Vbase=220000  Vref=1  Vangle=0  VLF=1  angleLF=0
      settings: AttributesFormatString=|
      | %<ID>
      | %<Vbase>V
      | %<VLF>pu
      | %<angleLF>deg.
      | %<Name>
  bus92 : powerlib/Measurements/Load Flow Bus  LConnTagsString=a  ID=bus92  Vbase=220000  Vref=1  Vangle=0  VLF=1  angleLF=0
      settings: AttributesFormatString=|
      | %<ID>
      | %<Vbase>V
      | %<VLF>pu
      | %<angleLF>deg.
      | %<Name>
  bus93 : powerlib/Measurements/Load Flow Bus  LConnTagsString=a  ID=bus93  Vbase=220000  Vref=1  Vangle=0  VLF=1  angleLF=0
      settings: AttributesFormatString=|
      | %<ID>
      | %<Vbase>V
      | %<VLF>pu
      | %<angleLF>deg.
      | %<Name>
  bus94 : powerlib/Measurements/Load Flow Bus  LConnTagsString=a  ID=bus94  Vbase=220000  Vref=1  Vangle=0  VLF=1  angleLF=0
      settings: AttributesFormatString=|
      | %<ID>
      | %<Vbase>V
      | %<VLF>pu
      | %<angleLF>deg.
      | %<Name>
  bus95 : powerlib/Measurements/Load Flow Bus  LConnTagsString=a  ID=bus95  Vbase=220000  Vref=1  Vangle=0  VLF=1  angleLF=0
      settings: AttributesFormatString=|
      | %<ID>
      | %<Vbase>V
      | %<VLF>pu
      | %<angleLF>deg.
      | %<Name>
  bus96 : powerlib/Measurements/Load Flow Bus  LConnTagsString=a  ID=bus96  Vbase=220000  Vref=1  Vangle=0  VLF=1  angleLF=0
      settings: AttributesFormatString=|
      | %<ID>
      | %<Vbase>V
      | %<VLF>pu
      | %<angleLF>deg.
      | %<Name>
  bus97 : powerlib/Measurements/Load Flow Bus  LConnTagsString=a  ID=bus97  Vbase=220000  Vref=1  Vangle=0  VLF=1  angleLF=0
      settings: AttributesFormatString=|
      | %<ID>
      | %<Vbase>V
      | %<VLF>pu
      | %<angleLF>deg.
      | %<Name>
  bus98 : powerlib/Measurements/Load Flow Bus  LConnTagsString=a  ID=bus98  Vbase=220000  Vref=1  Vangle=0  VLF=1  angleLF=0
      settings: AttributesFormatString=|
      | %<ID>
      | %<Vbase>V
      | %<VLF>pu
      | %<angleLF>deg.
      | %<Name>
  bus99 : powerlib/Measurements/Load Flow Bus  LConnTagsString=a  ID=bus99  Vbase=220000  Vref=1  Vangle=0  VLF=1  angleLF=0
      settings: AttributesFormatString=|
      | %<ID>
      | %<Vbase>V
      | %<VLF>pu
      | %<angleLF>deg.
      | %<Name>
  powergui : powerlib/powergui  Priority=1  SimulationMode=Continuous  SolverType=Tustin  SampleTime=50e-6  frequency=60  SPID=off  DisableSnubberDevices=off  DisableRonSwitches=off  DisableVfSwitches=off  SwTol=0  Interpol=off  DisplayEquations=off  Ts=0  methode=off  frequencyindice=60  Pbase=100e6  ErrMax=1e-4  Iterations=50  UnitsV=kV  UnitsW=MW  FunctionMessages=off  echomessages=off  HookPort=off  EnableUseOfTLC=off  x0status=blocks  RestoreLinks=warning  ResistiveCurrentMeasurement=off  Frange=[0:2:500]  Ylog=off  Xlog=on  ShowGrid=off  save=off  variable=ZData  structure=0  ZoomFFT=off  StartTime=0.0  cycles=1  DisplayStyle=1  fundamental=60  FreqAxis=off  MaxFrequency=1000  frequencyindicesteady=1  RmsSteady=1  display=off
  昌平一房山500kV紧_CN_275985691_500000_CN_276719460_500000 : powerlib/Elements/Distributed Parameters Line  Phases=3  Frequency=60  Resistance=[0.01273 0.3864]  Inductance="[0.9337e-3  4.1264e-3]"  Capacitance=[12.74e-9 7.751e-9]  Length=27.9626  x1=[0 0 0 0; 0.0001244 0 0 0; 0.0002488 0 0 0; 0.0003733 0 0 0; 0.0004977 0 0 0; 0.0006221 0 0 0]  x2=[0 0 0 0; 0.0001244 0 0 0; 0.0002488 0 0 0; 0.0003733 0 0 0; 0.0004977 0 0 0; 0.0006221 0 0 0]  x3=[0 0 0 0; 0.0001244 0 0 0; 0.0002488 0 0 0; 0.0003733 0 0 0; 0.0004977 0 0 0; 0.0006221 0 0 0]  x4=[0 0 0 0; 0.0001244 0 0 0; 0.0002488 0 0 0; 0.0003733 0 0 0; 0.0004977 0 0 0; 0.0006221 0 0 0]  x5=0  V1=ones(3,3)  V2=ones(3,3)  I1=ones(3,3)  I2=ones(3,3)  nHarmo=1  Measurements=None
  connections:
  _CN_105834287_110000_CN_121056846_110000/LConn1 -- T_105834287__/RConn1 -- _CN_105834287_110000_CN_287236841_110000/LConn1 -- L_105834287/LConn1
  _CN_105834287_110000_CN_121056846_110000/LConn2 -- T_105834287__/RConn2 -- _CN_105834287_110000_CN_287236841_110000/LConn2 -- L_105834287/LConn2
  _CN_105834287_110000_CN_121056846_110000/LConn3 -- T_105834287__/RConn3 -- _CN_105834287_110000_CN_287236841_110000/LConn3 -- L_105834287/LConn3 -- bus1/LConn1
  _CN_105834287_110000_CN_121056846_110000/RConn1 -- T_121056846__/LConn1 -- _CN_121056846_110000_CN_145499358_110000/LConn1
  _CN_105834287_110000_CN_121056846_110000/RConn2 -- T_121056846__/LConn2 -- _CN_121056846_110000_CN_145499358_110000/LConn2
  _CN_105834287_110000_CN_121056846_110000/RConn3 -- T_121056846__/LConn3 -- _CN_121056846_110000_CN_145499358_110000/LConn3 -- bus2/LConn1
  _CN_105834287_110000_CN_287236841_110000/RConn1 -- T_287236841__/RConn1 -- L_287236841/LConn1
  _CN_105834287_110000_CN_287236841_110000/RConn2 -- T_287236841__/RConn2 -- L_287236841/LConn2
  _CN_105834287_110000_CN_287236841_110000/RConn3 -- T_287236841__/RConn3 -- L_287236841/LConn3 -- bus3/LConn1
  _CN_121056846_110000_CN_145499358_110000/RConn1 -- T_145499358__/RConn1 -- _CN_145499354_110000_CN_145499358_110000/LConn1 -- _CN_145499355_110000_CN_145499358_110000/LConn1 -- _CN_145499356_110000_CN_145499358_110000/LConn1 -- L_145499358/LConn1
  _CN_121056846_110000_CN_145499358_110000/RConn2 -- T_145499358__/RConn2 -- _CN_145499354_110000_CN_145499358_110000/LConn2 -- _CN_145499355_110000_CN_145499358_110000/LConn2 -- _CN_145499356_110000_CN_145499358_110000/LConn2 -- L_145499358/LConn2
  _CN_121056846_110000_CN_145499358_110000/RConn3 -- T_145499358__/RConn3 -- _CN_145499354_110000_CN_145499358_110000/LConn3 -- _CN_145499355_110000_CN_145499358_110000/LConn3 -- _CN_145499356_110000_CN_145499358_110000/LConn3 -- L_145499358/LConn3 -- bus4/LConn1
  T_347775701_110000_110kV根亲变电站/LConn1 -- 110KV蓼杜线_CN_347775701_110000_CN_177340388_110000/LConn1
  T_347775701_110000_110kV根亲变电站/LConn2 -- 110KV蓼杜线_CN_347775701_110000_CN_177340388_110000/LConn2
  110KV蓼杜线_CN_347775701_110000_CN_177340388_110000/LConn3 -- T_347775701_110000_110kV根亲变电站/LConn3 -- bus5/LConn1
  T_177340388_110000_杜营110KV变电站/LConn1 -- 110KV蓼杜线_CN_347775701_110000_CN_177340388_110000/RConn1
  T_177340388_110000_杜营110KV变电站/LConn2 -- 110KV蓼杜线_CN_347775701_110000_CN_177340388_110000/RConn2
  110KV蓼杜线_CN_347775701_110000_CN_177340388_110000/RConn3 -- T_177340388_110000_杜营110KV变电站/LConn3 -- bus6/LConn1
  T_265301080_110000_/LConn1 -- _CN_265301080_110000_CN_275898479_110000/LConn1
  T_265301080_110000_/LConn2 -- _CN_265301080_110000_CN_275898479_110000/LConn2
  _CN_265301080_110000_CN_275898479_110000/LConn3 -- T_265301080_110000_/LConn3 -- bus7/LConn1
  _CN_265301080_110000_CN_275898479_110000/RConn1 -- T_275898479__/RConn1 -- _CN_136030445_110000_CN_275898479_110000/LConn1 -- L_275898479/LConn1
  _CN_265301080_110000_CN_275898479_110000/RConn2 -- T_275898479__/RConn2 -- _CN_136030445_110000_CN_275898479_110000/LConn2 -- L_275898479/LConn2
  _CN_265301080_110000_CN_275898479_110000/RConn3 -- T_275898479__/RConn3 -- _CN_136030445_110000_CN_275898479_110000/LConn3 -- L_275898479/LConn3 -- bus8/LConn1
  T_145499354__/LConn1 -- _CN_145499354_110000_CN_145499358_110000/RConn1
  T_145499354__/LConn2 -- _CN_145499354_110000_CN_145499358_110000/RConn2
  _CN_145499354_110000_CN_145499358_110000/RConn3 -- T_145499354__/LConn3 -- bus9/LConn1
  T_145499355__/LConn1 -- _CN_145499355_110000_CN_145499358_110000/RConn1
  T_145499355__/LConn2 -- _CN_145499355_110000_CN_145499358_110000/RConn2
  _CN_145499355_110000_CN_145499358_110000/RConn3 -- T_145499355__/LConn3 -- bus10/LConn1
  T_145499356__/LConn1 -- _CN_145499356_110000_CN_145499358_110000/RConn1
  T_145499356__/LConn2 -- _CN_145499356_110000_CN_145499358_110000/RConn2
  _CN_145499356_110000_CN_145499358_110000/RConn3 -- T_145499356__/LConn3 -- bus11/LConn1
  _CN_136030445_110000_CN_275898479_110000/RConn1 -- T_136030445_220000_/RConn1 -- L_136030445/LConn1
  _CN_136030445_110000_CN_275898479_110000/RConn2 -- T_136030445_220000_/RConn2 -- L_136030445/LConn2
  _CN_136030445_110000_CN_275898479_110000/RConn3 -- T_136030445_220000_/RConn3 -- L_136030445/LConn3 -- bus12/LConn1
  _CN_163985922_220000_CN_255311431_220000/LConn1 -- T_163985922__/RConn1 -- L_163985922/LConn1
  _CN_163985922_220000_CN_255311431_220000/LConn2 -- T_163985922__/RConn2 -- L_163985922/LConn2
  _CN_163985922_220000_CN_255311431_220000/LConn3 -- T_163985922__/RConn3 -- L_163985922/LConn3 -- bus13/LConn1
  _CN_163985922_220000_CN_255311431_220000/RConn1 -- T_255311431__/LConn1 -- _CN_255311430_220000_CN_255311431_220000/LConn1
  _CN_163985922_220000_CN_255311431_220000/RConn2 -- T_255311431__/LConn2 -- _CN_255311430_220000_CN_255311431_220000/LConn2
  _CN_163985922_220000_CN_255311431_220000/RConn3 -- T_255311431__/LConn3 -- _CN_255311430_220000_CN_255311431_220000/LConn3 -- bus14/LConn1
  _CN_161577477_220000_CN_278169207_220000/LConn1 -- T_161577477_220000_/LConn1 -- _CN_161577477_220000_CN_133523400_220000/LConn1
  _CN_161577477_220000_CN_278169207_220000/LConn2 -- T_161577477_220000_/LConn2 -- _CN_161577477_220000_CN_133523400_220000/LConn2
  _CN_161577477_220000_CN_278169207_220000/LConn3 -- T_161577477_220000_/LConn3 -- _CN_161577477_220000_CN_133523400_220000/LConn3 -- bus15/LConn1
  T_278169207__/LConn1 -- _CN_161577477_220000_CN_278169207_220000/RConn1
  T_278169207__/LConn2 -- _CN_161577477_220000_CN_278169207_220000/RConn2
  _CN_161577477_220000_CN_278169207_220000/RConn3 -- T_278169207__/LConn3 -- bus16/LConn1
  _CN_161577477_220000_CN_133523400_220000/RConn1 -- T_133523400_500000_/RConn1 -- _CN_321557804_220000_CN_133523400_220000/LConn1 -- L_133523400/LConn1
  _CN_161577477_220000_CN_133523400_220000/RConn2 -- T_133523400_500000_/RConn2 -- _CN_321557804_220000_CN_133523400_220000/LConn2 -- L_133523400/LConn2
  _CN_161577477_220000_CN_133523400_220000/RConn3 -- T_133523400_500000_/RConn3 -- _CN_321557804_220000_CN_133523400_220000/LConn3 -- L_133523400/LConn3 -- bus17/LConn1
  T_313629190_220000_/LConn1 -- _CN_313629190_220000_CN_315269978_220000/LConn1
  T_313629190_220000_/LConn2 -- _CN_313629190_220000_CN_315269978_220000/LConn2
  _CN_313629190_220000_CN_315269978_220000/LConn3 -- T_313629190_220000_/LConn3 -- bus18/LConn1
  T_315269978_220000_/LConn1 -- _CN_313629190_220000_CN_315269978_220000/RConn1
  T_315269978_220000_/LConn2 -- _CN_313629190_220000_CN_315269978_220000/RConn2
  _CN_313629190_220000_CN_315269978_220000/RConn3 -- T_315269978_220000_/LConn3 -- bus19/LConn1
  _CN_328518154_220000_CN_328842159_220000/LConn1 -- T_328518154_500000_/RConn1 -- L_328518154/LConn1
  _CN_328518154_220000_CN_328842159_220000/LConn2 -- T_328518154_500000_/RConn2 -- L_328518154/LConn2
  _CN_328518154_220000_CN_328842159_220000/LConn3 -- T_328518154_500000_/RConn3 -- L_328518154/LConn3 -- bus20/LConn1
  T_328842159_220000_/LConn1 -- _CN_328518154_220000_CN_328842159_220000/RConn1
  T_328842159_220000_/LConn2 -- _CN_328518154_220000_CN_328842159_220000/RConn2
  _CN_328518154_220000_CN_328842159_220000/RConn3 -- T_328842159_220000_/LConn3 -- bus21/LConn1
  _CN_284083287_220000_CN_284083294_220000/LConn1 -- T_284083287__/LConn1 -- _CN_284083287_220000_CN_284083280_220000/LConn1
  _CN_284083287_220000_CN_284083294_220000/LConn2 -- T_284083287__/LConn2 -- _CN_284083287_220000_CN_284083280_220000/LConn2
  _CN_284083287_220000_CN_284083294_220000/LConn3 -- T_284083287__/LConn3 -- _CN_284083287_220000_CN_284083280_220000/LConn3 -- bus22/LConn1
  T_284083294__/LConn1 -- _CN_284083287_220000_CN_284083294_220000/RConn1
  T_284083294__/LConn2 -- _CN_284083287_220000_CN_284083294_220000/RConn2
  _CN_284083287_220000_CN_284083294_220000/RConn3 -- T_284083294__/LConn3 -- bus23/LConn1
  T_284083280__/LConn1 -- _CN_284083287_220000_CN_284083280_220000/RConn1
  T_284083280__/LConn2 -- _CN_284083287_220000_CN_284083280_220000/RConn2
  _CN_284083287_220000_CN_284083280_220000/RConn3 -- T_284083280__/LConn3 -- bus24/LConn1
  _CN_315071500_220000_CN_315204024_220000/LConn1 -- T_315071500_500000_/RConn1 -- L_315071500/LConn1
  _CN_315071500_220000_CN_315204024_220000/LConn2 -- T_315071500_500000_/RConn2 -- L_315071500/LConn2
  _CN_315071500_220000_CN_315204024_220000/LConn3 -- T_315071500_500000_/RConn3 -- L_315071500/LConn3 -- bus25/LConn1
  T_315204024_220000_/LConn1 -- _CN_315071500_220000_CN_315204024_220000/RConn1
  T_315204024_220000_/LConn2 -- _CN_315071500_220000_CN_315204024_220000/RConn2
  _CN_315071500_220000_CN_315204024_220000/RConn3 -- T_315204024_220000_/LConn3 -- bus26/LConn1
  _CN_132443907_220000_CN_132430137_220000/LConn1 -- T_132443907__/RConn1 -- L_132443907/LConn1
  _CN_132443907_220000_CN_132430137_220000/LConn2 -- T_132443907__/RConn2 -- L_132443907/LConn2
  _CN_132443907_220000_CN_132430137_220000/LConn3 -- T_132443907__/RConn3 -- L_132443907/LConn3 -- bus27/LConn1
  _CN_132443907_220000_CN_132430137_220000/RConn1 -- T_132430137_500000_/RConn1 -- _CN_132503211_220000_CN_132430137_220000/LConn1 -- _CN_132430137_220000_CN_132312010_220000/LConn1 -- _CN_132430137_220000_CN_132312011_220000/LConn1 -- _CN_132430137_220000_CN_132430141_220000/LConn1 -- L_132430137/LConn1
  _CN_132443907_220000_CN_132430137_220000/RConn2 -- T_132430137_500000_/RConn2 -- _CN_132503211_220000_CN_132430137_220000/LConn2 -- _CN_132430137_220000_CN_132312010_220000/LConn2 -- _CN_132430137_220000_CN_132312011_220000/LConn2 -- _CN_132430137_220000_CN_132430141_220000/LConn2 -- L_132430137/LConn2
  _CN_132443907_220000_CN_132430137_220000/RConn3 -- T_132430137_500000_/RConn3 -- _CN_132503211_220000_CN_132430137_220000/LConn3 -- _CN_132430137_220000_CN_132312010_220000/LConn3 -- _CN_132430137_220000_CN_132312011_220000/LConn3 -- _CN_132430137_220000_CN_132430141_220000/LConn3 -- L_132430137/LConn3 -- bus28/LConn1
  _CN_150403605_220000_CN_127871762_220000/LConn1 -- T_150403605_220000_/LConn1 -- _CN_150403605_220000_CN_355642647_220000/LConn1
  _CN_150403605_220000_CN_127871762_220000/LConn2 -- T_150403605_220000_/LConn2 -- _CN_150403605_220000_CN_355642647_220000/LConn2
  _CN_150403605_220000_CN_127871762_220000/LConn3 -- T_150403605_220000_/LConn3 -- _CN_150403605_220000_CN_355642647_220000/LConn3 -- bus29/LConn1
  _CN_150403605_220000_CN_127871762_220000/RConn1 -- T_127871762_500000_/RConn1 -- L_127871762/LConn1
  _CN_150403605_220000_CN_127871762_220000/RConn2 -- T_127871762_500000_/RConn2 -- L_127871762/LConn2
  _CN_150403605_220000_CN_127871762_220000/RConn3 -- T_127871762_500000_/RConn3 -- L_127871762/LConn3 -- bus30/LConn1
  _CN_150403605_220000_CN_355642647_220000/RConn1 -- T_355642647__/LConn1 -- _CN_355642647_220000_CN_313585533_220000/LConn1 -- _CN_355642647_220000_CN_439464430_220000/LConn1
  _CN_150403605_220000_CN_355642647_220000/RConn2 -- T_355642647__/LConn2 -- _CN_355642647_220000_CN_313585533_220000/LConn2 -- _CN_355642647_220000_CN_439464430_220000/LConn2
  _CN_150403605_220000_CN_355642647_220000/RConn3 -- T_355642647__/LConn3 -- _CN_355642647_220000_CN_313585533_220000/LConn3 -- _CN_355642647_220000_CN_439464430_220000/LConn3 -- bus31/LConn1
  T_95783449__/LConn1 -- _CN_95783449_220000_CN_104955669_220000/LConn1
  T_95783449__/LConn2 -- _CN_95783449_220000_CN_104955669_220000/LConn2
  _CN_95783449_220000_CN_104955669_220000/LConn3 -- T_95783449__/LConn3 -- bus32/LConn1
  _CN_95783449_220000_CN_104955669_220000/RConn1 -- T_104955669__/LConn1 -- _CN_104955669_220000_CN_105894253_220000/LConn1 -- _CN_104955669_220000_CN_95513512_220000/LConn1
  _CN_95783449_220000_CN_104955669_220000/RConn2 -- T_104955669__/LConn2 -- _CN_104955669_220000_CN_105894253_220000/LConn2 -- _CN_104955669_220000_CN_95513512_220000/LConn2
  _CN_95783449_220000_CN_104955669_220000/RConn3 -- T_104955669__/LConn3 -- _CN_104955669_220000_CN_105894253_220000/LConn3 -- _CN_104955669_220000_CN_95513512_220000/LConn3 -- bus33/LConn1
  T_279415839__/LConn1 -- _CN_279415839_220000_CN_201195906_220000/LConn1
  T_279415839__/LConn2 -- _CN_279415839_220000_CN_201195906_220000/LConn2
  _CN_279415839_220000_CN_201195906_220000/LConn3 -- T_279415839__/LConn3 -- bus34/LConn1
  _CN_279415839_220000_CN_201195906_220000/RConn1 -- T_201195906_500000_/RConn1 -- _CN_201195906_220000_CN_201195907_220000/LConn1 -- L_201195906/LConn1
  _CN_279415839_220000_CN_201195906_220000/RConn2 -- T_201195906_500000_/RConn2 -- _CN_201195906_220000_CN_201195907_220000/LConn2 -- L_201195906/LConn2
  _CN_279415839_220000_CN_201195906_220000/RConn3 -- T_201195906_500000_/RConn3 -- _CN_201195906_220000_CN_201195907_220000/LConn3 -- L_201195906/LConn3 -- bus35/LConn1
  T_279415840__/LConn1 -- _CN_279415840_220000_CN_201197023_220000/LConn1
  T_279415840__/LConn2 -- _CN_279415840_220000_CN_201197023_220000/LConn2
  _CN_279415840_220000_CN_201197023_220000/LConn3 -- T_279415840__/LConn3 -- bus36/LConn1
  T_201197023_220000_/LConn1 -- _CN_279415840_220000_CN_201197023_220000/RConn1
  T_201197023_220000_/LConn2 -- _CN_279415840_220000_CN_201197023_220000/RConn2
  _CN_279415840_220000_CN_201197023_220000/RConn3 -- T_201197023_220000_/LConn3 -- bus37/LConn1
  _CN_275706404_220000_CN_275706430_220000/LConn1 -- T_275706404__/LConn1 -- _CN_275706404_220000_CN_276589707_220000/LConn1
  _CN_275706404_220000_CN_275706430_220000/LConn2 -- T_275706404__/LConn2 -- _CN_275706404_220000_CN_276589707_220000/LConn2
  _CN_275706404_220000_CN_275706430_220000/LConn3 -- T_275706404__/LConn3 -- _CN_275706404_220000_CN_276589707_220000/LConn3 -- bus38/LConn1
  _CN_275706404_220000_CN_275706430_220000/RConn1 -- T_275706430_500000_昌平变电站/RConn1 -- _CN_275706430_220000_CN_330370369_220000/LConn1 -- L_275706430/LConn1
  _CN_275706404_220000_CN_275706430_220000/RConn2 -- T_275706430_500000_昌平变电站/RConn2 -- _CN_275706430_220000_CN_330370369_220000/LConn2 -- L_275706430/LConn2
  _CN_275706404_220000_CN_275706430_220000/RConn3 -- T_275706430_500000_昌平变电站/RConn3 -- _CN_275706430_220000_CN_330370369_220000/LConn3 -- L_275706430/LConn3 -- bus39/LConn1
  T_276589707__/LConn1 -- _CN_275706404_220000_CN_276589707_220000/RConn1
  T_276589707__/LConn2 -- _CN_275706404_220000_CN_276589707_220000/RConn2
  _CN_275706404_220000_CN_276589707_220000/RConn3 -- T_276589707__/LConn3 -- bus40/LConn1
  T_119206438_220000_/LConn1 -- _CN_119206438_220000_CN_119206440_220000/LConn1
  T_119206438_220000_/LConn2 -- _CN_119206438_220000_CN_119206440_220000/LConn2
  _CN_119206438_220000_CN_119206440_220000/LConn3 -- T_119206438_220000_/LConn3 -- bus41/LConn1
  _CN_119206438_220000_CN_119206440_220000/RConn1 -- T_119206440_220000_/LConn1 -- _CN_119206440_220000_CN_223806191_220000/LConn1
  _CN_119206438_220000_CN_119206440_220000/RConn2 -- T_119206440_220000_/LConn2 -- _CN_119206440_220000_CN_223806191_220000/LConn2
  _CN_119206438_220000_CN_119206440_220000/RConn3 -- T_119206440_220000_/LConn3 -- _CN_119206440_220000_CN_223806191_220000/LConn3 -- bus42/LConn1
  T_223806191_220000_/LConn1 -- _CN_119206440_220000_CN_223806191_220000/RConn1
  T_223806191_220000_/LConn2 -- _CN_119206440_220000_CN_223806191_220000/RConn2
  _CN_119206440_220000_CN_223806191_220000/RConn3 -- T_223806191_220000_/LConn3 -- bus43/LConn1
  T_279419433__/LConn1 -- _CN_279419433_220000_CN_135466215_220000/LConn1
  T_279419433__/LConn2 -- _CN_279419433_220000_CN_135466215_220000/LConn2
  _CN_279419433_220000_CN_135466215_220000/LConn3 -- T_279419433__/LConn3 -- bus44/LConn1
  _CN_279419433_220000_CN_135466215_220000/RConn1 -- T_135466215_500000_天津北郊/RConn1 -- _CN_264823742_220000_CN_135466215_220000/LConn1 -- L_135466215/LConn1
  _CN_279419433_220000_CN_135466215_220000/RConn2 -- T_135466215_500000_天津北郊/RConn2 -- _CN_264823742_220000_CN_135466215_220000/LConn2 -- L_135466215/LConn2
  _CN_279419433_220000_CN_135466215_220000/RConn3 -- T_135466215_500000_天津北郊/RConn3 -- _CN_264823742_220000_CN_135466215_220000/LConn3 -- L_135466215/LConn3 -- bus45/LConn1
  T_162378077__/LConn1 -- _CN_162378077_220000_CN_162378099_220000/LConn1
  T_162378077__/LConn2 -- _CN_162378077_220000_CN_162378099_220000/LConn2
  _CN_162378077_220000_CN_162378099_220000/LConn3 -- T_162378077__/LConn3 -- bus46/LConn1
  _CN_162378077_220000_CN_162378099_220000/RConn1 -- T_162378099__/LConn1 -- _CN_162167607_220000_CN_162378099_220000/LConn1
  _CN_162378077_220000_CN_162378099_220000/RConn2 -- T_162378099__/LConn2 -- _CN_162167607_220000_CN_162378099_220000/LConn2
  _CN_162378077_220000_CN_162378099_220000/RConn3 -- T_162378099__/LConn3 -- _CN_162167607_220000_CN_162378099_220000/LConn3 -- bus47/LConn1
  T_285846074__/LConn1 -- _CN_285846074_220000_CN_145499358_220000/LConn1
  T_285846074__/LConn2 -- _CN_285846074_220000_CN_145499358_220000/LConn2
  _CN_285846074_220000_CN_145499358_220000/LConn3 -- T_285846074__/LConn3 -- bus48/LConn1
  _CN_285846074_220000_CN_145499358_220000/RConn1 -- T_145499358__/LConn1 -- _CN_145499358_220000_CN_121056862_220000/LConn1
  _CN_285846074_220000_CN_145499358_220000/RConn2 -- T_145499358__/LConn2 -- _CN_145499358_220000_CN_121056862_220000/LConn2
  _CN_285846074_220000_CN_145499358_220000/RConn3 -- T_145499358__/LConn3 -- _CN_145499358_220000_CN_121056862_220000/LConn3 -- bus49/LConn1
  _CN_107025759_220000_CN_287591085_220000/LConn1 -- T_107025759_220000_/LConn1 -- _CN_107025759_220000_CN_95805677_220000/LConn1
  _CN_107025759_220000_CN_287591085_220000/LConn2 -- T_107025759_220000_/LConn2 -- _CN_107025759_220000_CN_95805677_220000/LConn2
  _CN_107025759_220000_CN_287591085_220000/LConn3 -- T_107025759_220000_/LConn3 -- _CN_107025759_220000_CN_95805677_220000/LConn3 -- bus50/LConn1
  _CN_107025759_220000_CN_287591085_220000/RConn1 -- T_287591085_500000_国家电网500千伏特高压练塘变电站/RConn1 -- L_287591085/LConn1
  _CN_107025759_220000_CN_287591085_220000/RConn2 -- T_287591085_500000_国家电网500千伏特高压练塘变电站/RConn2 -- L_287591085/LConn2
  _CN_107025759_220000_CN_287591085_220000/RConn3 -- T_287591085_500000_国家电网500千伏特高压练塘变电站/RConn3 -- L_287591085/LConn3 -- bus51/LConn1
  _CN_107025759_220000_CN_95805677_220000/RConn1 -- T_95805677_500000_/RConn1 -- _CN_107081079_220000_CN_95805677_220000/LConn1 -- L_95805677/LConn1 -- _CN_107025734_220000_CN_95805677_220000/LConn1 -- _CN_107025757_220000_CN_95805677_220000/LConn1 -- _CN_95801089_220000_CN_95805677_220000/LConn1 -- _CN_106027291_220000_CN_95805677_220000/LConn1
  _CN_107025759_220000_CN_95805677_220000/RConn2 -- T_95805677_500000_/RConn2 -- _CN_107081079_220000_CN_95805677_220000/LConn2 -- L_95805677/LConn2 -- _CN_107025734_220000_CN_95805677_220000/LConn2 -- _CN_107025757_220000_CN_95805677_220000/LConn2 -- _CN_95801089_220000_CN_95805677_220000/LConn2 -- _CN_106027291_220000_CN_95805677_220000/LConn2
  _CN_107025759_220000_CN_95805677_220000/RConn3 -- T_95805677_500000_/RConn3 -- _CN_107081079_220000_CN_95805677_220000/LConn3 -- L_95805677/LConn3 -- bus52/LConn1 -- _CN_107025734_220000_CN_95805677_220000/LConn3 -- _CN_107025757_220000_CN_95805677_220000/LConn3 -- _CN_95801089_220000_CN_95805677_220000/LConn3 -- _CN_106027291_220000_CN_95805677_220000/LConn3
  T_330370369__/LConn1 -- _CN_275706430_220000_CN_330370369_220000/RConn1
  T_330370369__/LConn2 -- _CN_275706430_220000_CN_330370369_220000/RConn2
  _CN_275706430_220000_CN_330370369_220000/RConn3 -- T_330370369__/LConn3 -- bus53/LConn1
  T_95783487__/LConn1 -- _CN_95783487_220000_CN_95783492_220000/LConn1
  T_95783487__/LConn2 -- _CN_95783487_220000_CN_95783492_220000/LConn2
  _CN_95783487_220000_CN_95783492_220000/LConn3 -- T_95783487__/LConn3 -- bus54/LConn1
  _CN_95783487_220000_CN_95783492_220000/RConn1 -- T_95783492__/LConn1 -- _CN_95783492_220000_CN_95093839_220000/LConn1 -- _CN_95783492_220000_CN_95783495_220000/LConn1 -- _CN_95783492_220000_CN_95513512_220000/LConn1
  _CN_95783487_220000_CN_95783492_220000/RConn2 -- T_95783492__/LConn2 -- _CN_95783492_220000_CN_95093839_220000/LConn2 -- _CN_95783492_220000_CN_95783495_220000/LConn2 -- _CN_95783492_220000_CN_95513512_220000/LConn2
  _CN_95783487_220000_CN_95783492_220000/RConn3 -- T_95783492__/LConn3 -- _CN_95783492_220000_CN_95093839_220000/LConn3 -- _CN_95783492_220000_CN_95783495_220000/LConn3 -- _CN_95783492_220000_CN_95513512_220000/LConn3 -- bus55/LConn1
  T_284039744__/LConn1 -- _CN_284039744_220000_CN_283658134_220000/LConn1
  T_284039744__/LConn2 -- _CN_284039744_220000_CN_283658134_220000/LConn2
  _CN_284039744_220000_CN_283658134_220000/LConn3 -- T_284039744__/LConn3 -- bus56/LConn1
  _CN_284039744_220000_CN_283658134_220000/RConn1 -- T_283658134__/RConn1 -- L_283658134/LConn1
  _CN_284039744_220000_CN_283658134_220000/RConn2 -- T_283658134__/RConn2 -- L_283658134/LConn2
  _CN_284039744_220000_CN_283658134_220000/RConn3 -- T_283658134__/RConn3 -- L_283658134/LConn3 -- bus57/LConn1
  _CN_147744835_220000_CN_188973331_220000/LConn1 -- T_147744835_500000_/RConn1 -- _CN_147744835_220000_CN_188829044_220000/LConn1 -- L_147744835/LConn1
  _CN_147744835_220000_CN_188973331_220000/LConn2 -- T_147744835_500000_/RConn2 -- _CN_147744835_220000_CN_188829044_220000/LConn2 -- L_147744835/LConn2
  _CN_147744835_220000_CN_188973331_220000/LConn3 -- T_147744835_500000_/RConn3 -- _CN_147744835_220000_CN_188829044_220000/LConn3 -- L_147744835/LConn3 -- bus58/LConn1
  T_188973331_220000_/LConn1 -- _CN_147744835_220000_CN_188973331_220000/RConn1
  T_188973331_220000_/LConn2 -- _CN_147744835_220000_CN_188973331_220000/RConn2
  _CN_147744835_220000_CN_188973331_220000/RConn3 -- T_188973331_220000_/LConn3 -- bus59/LConn1
  _CN_147744835_220000_CN_188829044_220000/RConn1 -- T_188829044_500000_/RConn1 -- _CN_189931119_220000_CN_188829044_220000/LConn1 -- L_188829044/LConn1
  _CN_147744835_220000_CN_188829044_220000/RConn2 -- T_188829044_500000_/RConn2 -- _CN_189931119_220000_CN_188829044_220000/LConn2 -- L_188829044/LConn2
  _CN_147744835_220000_CN_188829044_220000/RConn3 -- T_188829044_500000_/RConn3 -- _CN_189931119_220000_CN_188829044_220000/LConn3 -- L_188829044/LConn3 -- bus60/LConn1
  _CN_95783492_220000_CN_95093839_220000/RConn1 -- T_95093839__/LConn1 -- _CN_95093839_220000_CN_106027291_220000/LConn1
  _CN_95783492_220000_CN_95093839_220000/RConn2 -- T_95093839__/LConn2 -- _CN_95093839_220000_CN_106027291_220000/LConn2
  _CN_95783492_220000_CN_95093839_220000/RConn3 -- T_95093839__/LConn3 -- _CN_95093839_220000_CN_106027291_220000/LConn3 -- bus61/LConn1
  _CN_95783492_220000_CN_95783495_220000/RConn1 -- T_95783495__/LConn1 -- _CN_95783495_220000_CN_95783496_220000/LConn1
  _CN_95783492_220000_CN_95783495_220000/RConn2 -- T_95783495__/LConn2 -- _CN_95783495_220000_CN_95783496_220000/LConn2
  _CN_95783492_220000_CN_95783495_220000/RConn3 -- T_95783495__/LConn3 -- _CN_95783495_220000_CN_95783496_220000/LConn3 -- bus62/LConn1
  _CN_95783492_220000_CN_95513512_220000/RConn1 -- T_95513512__/LConn1 -- _CN_106027291_220000_CN_95513512_220000/LConn1 -- _CN_104955669_220000_CN_95513512_220000/RConn1
  _CN_95783492_220000_CN_95513512_220000/RConn2 -- T_95513512__/LConn2 -- _CN_106027291_220000_CN_95513512_220000/LConn2 -- _CN_104955669_220000_CN_95513512_220000/RConn2
  _CN_95783492_220000_CN_95513512_220000/RConn3 -- T_95513512__/LConn3 -- _CN_106027291_220000_CN_95513512_220000/LConn3 -- bus63/LConn1 -- _CN_104955669_220000_CN_95513512_220000/RConn3
  T_255311430__/LConn1 -- _CN_255311430_220000_CN_255311431_220000/RConn1
  T_255311430__/LConn2 -- _CN_255311430_220000_CN_255311431_220000/RConn2
  _CN_255311430_220000_CN_255311431_220000/RConn3 -- T_255311430__/LConn3 -- bus64/LConn1
  T_95783496__/LConn1 -- _CN_95783495_220000_CN_95783496_220000/RConn1
  T_95783496__/LConn2 -- _CN_95783495_220000_CN_95783496_220000/RConn2
  _CN_95783495_220000_CN_95783496_220000/RConn3 -- T_95783496__/LConn3 -- bus65/LConn1
  T_284083277__/LConn1 -- _CN_284083277_220000_CN_284083293_220000/LConn1
  T_284083277__/LConn2 -- _CN_284083277_220000_CN_284083293_220000/LConn2
  _CN_284083277_220000_CN_284083293_220000/LConn3 -- T_284083277__/LConn3 -- bus66/LConn1
  _CN_284083277_220000_CN_284083293_220000/RConn1 -- T_284083293__/LConn1 -- _CN_284083293_220000_CN_283658122_220000/LConn1
  _CN_284083277_220000_CN_284083293_220000/RConn2 -- T_284083293__/LConn2 -- _CN_284083293_220000_CN_283658122_220000/LConn2
  _CN_284083277_220000_CN_284083293_220000/RConn3 -- T_284083293__/LConn3 -- _CN_284083293_220000_CN_283658122_220000/LConn3 -- bus67/LConn1
  _CN_95093839_220000_CN_106027291_220000/RConn1 -- T_106027291_500000_/RConn1 -- _CN_106027291_220000_CN_95805677_220000/RConn1 -- _CN_106027291_220000_CN_95513512_220000/RConn1 -- L_106027291/LConn1
  _CN_95093839_220000_CN_106027291_220000/RConn2 -- T_106027291_500000_/RConn2 -- _CN_106027291_220000_CN_95805677_220000/RConn2 -- _CN_106027291_220000_CN_95513512_220000/RConn2 -- L_106027291/LConn2
  _CN_95093839_220000_CN_106027291_220000/RConn3 -- T_106027291_500000_/RConn3 -- _CN_106027291_220000_CN_95805677_220000/RConn3 -- _CN_106027291_220000_CN_95513512_220000/RConn3 -- L_106027291/LConn3 -- bus68/LConn1
  T_225119562__/LConn1 -- _CN_225119562_220000_CN_314606534_220000/LConn1
  T_225119562__/LConn2 -- _CN_225119562_220000_CN_314606534_220000/LConn2
  _CN_225119562_220000_CN_314606534_220000/LConn3 -- T_225119562__/LConn3 -- bus69/LConn1
  T_314606534_220000_/LConn1 -- _CN_225119562_220000_CN_314606534_220000/RConn1
  T_314606534_220000_/LConn2 -- _CN_225119562_220000_CN_314606534_220000/RConn2
  _CN_225119562_220000_CN_314606534_220000/RConn3 -- T_314606534_220000_/LConn3 -- bus70/LConn1
  T_147710033_220000_/LConn1 -- _CN_147710033_220000_CN_147708063_220000/LConn1
  T_147710033_220000_/LConn2 -- _CN_147710033_220000_CN_147708063_220000/LConn2
  _CN_147710033_220000_CN_147708063_220000/LConn3 -- T_147710033_220000_/LConn3 -- bus71/LConn1
  _CN_147710033_220000_CN_147708063_220000/RConn1 -- T_147708063_500000_/RConn1 -- _CN_147706495_220000_CN_147708063_220000/LConn1 -- _CN_189145223_220000_CN_147708063_220000/LConn1 -- _CN_147708063_220000_CN_189139925_220000/LConn1 -- L_147708063/LConn1
  _CN_147710033_220000_CN_147708063_220000/RConn2 -- T_147708063_500000_/RConn2 -- _CN_147706495_220000_CN_147708063_220000/LConn2 -- _CN_189145223_220000_CN_147708063_220000/LConn2 -- _CN_147708063_220000_CN_189139925_220000/LConn2 -- L_147708063/LConn2
  _CN_147710033_220000_CN_147708063_220000/RConn3 -- T_147708063_500000_/RConn3 -- _CN_147706495_220000_CN_147708063_220000/LConn3 -- _CN_189145223_220000_CN_147708063_220000/LConn3 -- _CN_147708063_220000_CN_189139925_220000/LConn3 -- L_147708063/LConn3 -- bus72/LConn1
  _CN_280851769_220000_CN_136030445_220000/LConn1 -- T_280851769__/LConn1 -- _CN_280851769_220000_CN_275898479_220000/LConn1
  _CN_280851769_220000_CN_136030445_220000/LConn2 -- T_280851769__/LConn2 -- _CN_280851769_220000_CN_275898479_220000/LConn2
  _CN_280851769_220000_CN_136030445_220000/LConn3 -- T_280851769__/LConn3 -- _CN_280851769_220000_CN_275898479_220000/LConn3 -- bus73/LConn1
  _CN_280851769_220000_CN_136030445_220000/RConn1 -- T_136030445_220000_/LConn1 -- _CN_275898479_220000_CN_136030445_220000/LConn1
  _CN_280851769_220000_CN_136030445_220000/RConn2 -- T_136030445_220000_/LConn2 -- _CN_275898479_220000_CN_136030445_220000/LConn2
  _CN_280851769_220000_CN_136030445_220000/RConn3 -- T_136030445_220000_/LConn3 -- _CN_275898479_220000_CN_136030445_220000/LConn3 -- bus74/LConn1
  _CN_280851769_220000_CN_275898479_220000/RConn1 -- T_275898479__/LConn1 -- _CN_275898479_220000_CN_136030445_220000/RConn1
  _CN_280851769_220000_CN_275898479_220000/RConn2 -- T_275898479__/LConn2 -- _CN_275898479_220000_CN_136030445_220000/RConn2
  _CN_280851769_220000_CN_275898479_220000/RConn3 -- T_275898479__/LConn3 -- _CN_275898479_220000_CN_136030445_220000/RConn3 -- bus75/LConn1
  T_323016549_500000_/LConn1 -- _CN_323016549_220000_CN_323106411_220000/LConn1
  T_323016549_500000_/LConn2 -- _CN_323016549_220000_CN_323106411_220000/LConn2
  _CN_323016549_220000_CN_323106411_220000/LConn3 -- T_323016549_500000_/LConn3 -- bus76/LConn1
  _CN_323016549_220000_CN_323106411_220000/RConn1 -- T_323106411_220000_/RConn1 -- _CN_323106411_220000_CN_323106340_220000/LConn1 -- L_323106411/LConn1
  _CN_323016549_220000_CN_323106411_220000/RConn2 -- T_323106411_220000_/RConn2 -- _CN_323106411_220000_CN_323106340_220000/LConn2 -- L_323106411/LConn2
  _CN_323016549_220000_CN_323106411_220000/RConn3 -- T_323106411_220000_/RConn3 -- _CN_323106411_220000_CN_323106340_220000/LConn3 -- L_323106411/LConn3 -- bus77/LConn1
  _CN_128686690_220000_CN_128731546_220000/LConn1 -- T_128686690_500000_/RConn1 -- _CN_128686690_220000_CN_171484817_220000/LConn1 -- L_128686690/LConn1
  _CN_128686690_220000_CN_128731546_220000/LConn2 -- T_128686690_500000_/RConn2 -- _CN_128686690_220000_CN_171484817_220000/LConn2 -- L_128686690/LConn2
  _CN_128686690_220000_CN_128731546_220000/LConn3 -- T_128686690_500000_/RConn3 -- _CN_128686690_220000_CN_171484817_220000/LConn3 -- L_128686690/LConn3 -- bus78/LConn1
  _CN_128686690_220000_CN_128731546_220000/RConn1 -- T_128731546__/LConn1 -- _CN_128731545_220000_CN_128731546_220000/LConn1
  _CN_128686690_220000_CN_128731546_220000/RConn2 -- T_128731546__/LConn2 -- _CN_128731545_220000_CN_128731546_220000/LConn2
  _CN_128686690_220000_CN_128731546_220000/RConn3 -- T_128731546__/LConn3 -- _CN_128731545_220000_CN_128731546_220000/LConn3 -- bus79/LConn1
  T_171484817__/LConn1 -- _CN_128686690_220000_CN_171484817_220000/RConn1
  T_171484817__/LConn2 -- _CN_128686690_220000_CN_171484817_220000/RConn2
  _CN_128686690_220000_CN_171484817_220000/RConn3 -- T_171484817__/LConn3 -- bus80/LConn1
  T_170221358_220000_/LConn1 -- _CN_170221358_220000_CN_170206555_220000/LConn1
  T_170221358_220000_/LConn2 -- _CN_170221358_220000_CN_170206555_220000/LConn2
  _CN_170221358_220000_CN_170206555_220000/LConn3 -- T_170221358_220000_/LConn3 -- bus81/LConn1
  _CN_170221358_220000_CN_170206555_220000/RConn1 -- T_170206555_500000_Pengzhou_Substation/LConn1 -- _CN_170216134_220000_CN_170206555_220000/LConn1
  _CN_170221358_220000_CN_170206555_220000/RConn2 -- T_170206555_500000_Pengzhou_Substation/LConn2 -- _CN_170216134_220000_CN_170206555_220000/LConn2
  _CN_170221358_220000_CN_170206555_220000/RConn3 -- T_170206555_500000_Pengzhou_Substation/LConn3 -- _CN_170216134_220000_CN_170206555_220000/LConn3 -- bus82/LConn1
  _CN_259721828_220000_CN_328639863_220000/LConn1 -- T_259721828_500000_/RConn1 -- L_259721828/LConn1
  _CN_259721828_220000_CN_328639863_220000/LConn2 -- T_259721828_500000_/RConn2 -- L_259721828/LConn2
  _CN_259721828_220000_CN_328639863_220000/LConn3 -- T_259721828_500000_/RConn3 -- L_259721828/LConn3 -- bus83/LConn1
  T_328639863__/LConn1 -- _CN_259721828_220000_CN_328639863_220000/RConn1
  T_328639863__/LConn2 -- _CN_259721828_220000_CN_328639863_220000/RConn2
  _CN_259721828_220000_CN_328639863_220000/RConn3 -- T_328639863__/LConn3 -- bus84/LConn1
  _CN_313528427_220000_CN_313585532_220000/LConn1 -- T_313528427_500000_/RConn1 -- L_313528427/LConn1
  _CN_313528427_220000_CN_313585532_220000/LConn2 -- T_313528427_500000_/RConn2 -- L_313528427/LConn2
  _CN_313528427_220000_CN_313585532_220000/LConn3 -- T_313528427_500000_/RConn3 -- L_313528427/LConn3 -- bus85/LConn1
  _CN_313528427_220000_CN_313585532_220000/RConn1 -- T_313585532_220000_/LConn1 -- _CN_313585532_220000_CN_313585533_220000/LConn1
  _CN_313528427_220000_CN_313585532_220000/RConn2 -- T_313585532_220000_/LConn2 -- _CN_313585532_220000_CN_313585533_220000/LConn2
  _CN_313528427_220000_CN_313585532_220000/RConn3 -- T_313585532_220000_/LConn3 -- _CN_313585532_220000_CN_313585533_220000/LConn3 -- bus86/LConn1
  T_312852588__/LConn1 -- _CN_312852588_220000_CN_312852605_220000/LConn1
  T_312852588__/LConn2 -- _CN_312852588_220000_CN_312852605_220000/LConn2
  _CN_312852588_220000_CN_312852605_220000/LConn3 -- T_312852588__/LConn3 -- bus87/LConn1
  _CN_312852588_220000_CN_312852605_220000/RConn1 -- T_312852605__/LConn1 -- _CN_312852605_220000_CN_277704920_220000/LConn1
  _CN_312852588_220000_CN_312852605_220000/RConn2 -- T_312852605__/LConn2 -- _CN_312852605_220000_CN_277704920_220000/LConn2
  _CN_312852588_220000_CN_312852605_220000/RConn3 -- T_312852605__/LConn3 -- _CN_312852605_220000_CN_277704920_220000/LConn3 -- bus88/LConn1
  _CN_148727570_220000_CN_279595711_220000/LConn1 -- T_148727570_500000_/RConn1 -- _CN_148727570_220000_CN_278530118_220000/LConn1 -- L_148727570/LConn1
  _CN_148727570_220000_CN_279595711_220000/LConn2 -- T_148727570_500000_/RConn2 -- _CN_148727570_220000_CN_278530118_220000/LConn2 -- L_148727570/LConn2
  _CN_148727570_220000_CN_279595711_220000/LConn3 -- T_148727570_500000_/RConn3 -- _CN_148727570_220000_CN_278530118_220000/LConn3 -- L_148727570/LConn3 -- bus89/LConn1
  _CN_148727570_220000_CN_279595711_220000/RConn1 -- T_279595711__/LConn1 -- _CN_279595711_220000_CN_312789337_220000/LConn1
  _CN_148727570_220000_CN_279595711_220000/RConn2 -- T_279595711__/LConn2 -- _CN_279595711_220000_CN_312789337_220000/LConn2
  _CN_148727570_220000_CN_279595711_220000/RConn3 -- T_279595711__/LConn3 -- _CN_279595711_220000_CN_312789337_220000/LConn3 -- bus90/LConn1
  T_278530118__/LConn1 -- _CN_148727570_220000_CN_278530118_220000/RConn1
  T_278530118__/LConn2 -- _CN_148727570_220000_CN_278530118_220000/RConn2
  _CN_148727570_220000_CN_278530118_220000/RConn3 -- T_278530118__/LConn3 -- bus91/LConn1
  T_189931119__/LConn1 -- _CN_189931119_220000_CN_188829044_220000/RConn1
  T_189931119__/LConn2 -- _CN_189931119_220000_CN_188829044_220000/RConn2
  _CN_189931119_220000_CN_188829044_220000/RConn3 -- T_189931119__/LConn3 -- bus92/LConn1
  T_319534355__/LConn1 -- _CN_319534355_220000_CN_314288467_220000/LConn1
  T_319534355__/LConn2 -- _CN_319534355_220000_CN_314288467_220000/LConn2
  _CN_319534355_220000_CN_314288467_220000/LConn3 -- T_319534355__/LConn3 -- bus93/LConn1
  _CN_319534355_220000_CN_314288467_220000/RConn1 -- T_314288467_500000_/RConn1 -- _CN_314318262_220000_CN_314288467_220000/LConn1 -- L_314288467/LConn1
  _CN_319534355_220000_CN_314288467_220000/RConn2 -- T_314288467_500000_/RConn2 -- _CN_314318262_220000_CN_314288467_220000/LConn2 -- L_314288467/LConn2
  _CN_319534355_220000_CN_314288467_220000/RConn3 -- T_314288467_500000_/RConn3 -- _CN_314318262_220000_CN_314288467_220000/LConn3 -- L_314288467/LConn3 -- bus94/LConn1
  _CN_365846132_220000_CN_136348806_220000/LConn1 -- T_365846132__/LConn1 -- _CN_365846132_220000_CN_277880965_220000/LConn1
  _CN_365846132_220000_CN_136348806_220000/LConn2 -- T_365846132__/LConn2 -- _CN_365846132_220000_CN_277880965_220000/LConn2
  _CN_365846132_220000_CN_136348806_220000/LConn3 -- T_365846132__/LConn3 -- _CN_365846132_220000_CN_277880965_220000/LConn3 -- bus95/LConn1
  _CN_365846132_220000_CN_136348806_220000/RConn1 -- T_136348806_500000_/RConn1 -- _CN_136348806_220000_CN_258077674_220000/LConn1 -- _CN_136348806_220000_CN_279442214_220000/LConn1 -- L_136348806/LConn1
  _CN_365846132_220000_CN_136348806_220000/RConn2 -- T_136348806_500000_/RConn2 -- _CN_136348806_220000_CN_258077674_220000/LConn2 -- _CN_136348806_220000_CN_279442214_220000/LConn2 -- L_136348806/LConn2
  _CN_365846132_220000_CN_136348806_220000/RConn3 -- T_136348806_500000_/RConn3 -- _CN_136348806_220000_CN_258077674_220000/LConn3 -- _CN_136348806_220000_CN_279442214_220000/LConn3 -- L_136348806/LConn3 -- bus96/LConn1
  _CN_365846132_220000_CN_277880965_220000/RConn1 -- T_277880965__/LConn1 -- _CN_277880965_220000_CN_365843497_220000/LConn1
  _CN_365846132_220000_CN_277880965_220000/RConn2 -- T_277880965__/LConn2 -- _CN_277880965_220000_CN_365843497_220000/LConn2
  _CN_365846132_220000_CN_277880965_220000/RConn3 -- T_277880965__/LConn3 -- _CN_277880965_220000_CN_365843497_220000/LConn3 -- bus97/LConn1
  _CN_264823742_220000_CN_135466215_220000/RConn1 -- T_264823742_220000_/LConn1 -- _CN_264823742_220000_CN_282759079_220000/LConn1
  _CN_264823742_220000_CN_135466215_220000/RConn2 -- T_264823742_220000_/LConn2 -- _CN_264823742_220000_CN_282759079_220000/LConn2
  _CN_264823742_220000_CN_135466215_220000/RConn3 -- T_264823742_220000_/LConn3 -- _CN_264823742_220000_CN_282759079_220000/LConn3 -- bus98/LConn1
  T_282759079__/LConn1 -- _CN_264823742_220000_CN_282759079_220000/RConn1
  T_282759079__/LConn2 -- _CN_264823742_220000_CN_282759079_220000/RConn2
  _CN_264823742_220000_CN_282759079_220000/RConn3 -- T_282759079__/LConn3 -- bus99/LConn1
  T_284477051__/LConn1 -- _CN_284477051_220000_CN_100600532_220000/LConn1
  T_284477051__/LConn2 -- _CN_284477051_220000_CN_100600532_220000/LConn2
  _CN_284477051_220000_CN_100600532_220000/LConn3 -- T_284477051__/LConn3 -- bus100/LConn1
  _CN_284477051_220000_CN_100600532_220000/RConn1 -- T_100600532__/RConn1 -- L_100600532/LConn1
  _CN_284477051_220000_CN_100600532_220000/RConn2 -- T_100600532__/RConn2 -- L_100600532/LConn2
  _CN_284477051_220000_CN_100600532_220000/RConn3 -- T_100600532__/RConn3 -- L_100600532/LConn3 -- bus101/LConn1
  _CN_312852604_220000_CN_278062434_220000/LConn1 -- T_312852604__/LConn1 -- _CN_312852604_220000_CN_277499262_220000/LConn1
  _CN_312852604_220000_CN_278062434_220000/LConn2 -- T_312852604__/LConn2 -- _CN_312852604_220000_CN_277499262_220000/LConn2
  _CN_312852604_220000_CN_278062434_220000/LConn3 -- T_312852604__/LConn3 -- _CN_312852604_220000_CN_277499262_220000/LConn3 -- bus102/LConn1
  T_278062434__/LConn1 -- _CN_312852604_220000_CN_278062434_220000/RConn1
  T_278062434__/LConn2 -- _CN_312852604_220000_CN_278062434_220000/RConn2
  _CN_312852604_220000_CN_278062434_220000/RConn3 -- T_278062434__/LConn3 -- bus103/LConn1
  _CN_312852604_220000_CN_277499262_220000/RConn1 -- T_277499262__/RConn1 -- _CN_279711874_220000_CN_277499262_220000/LConn1 -- L_277499262/LConn1
  _CN_312852604_220000_CN_277499262_220000/RConn2 -- T_277499262__/RConn2 -- _CN_279711874_220000_CN_277499262_220000/LConn2 -- L_277499262/LConn2
  _CN_312852604_220000_CN_277499262_220000/RConn3 -- T_277499262__/RConn3 -- _CN_279711874_220000_CN_277499262_220000/LConn3 -- L_277499262/LConn3 -- bus104/LConn1
  _CN_312852605_220000_CN_277704920_220000/RConn1 -- T_277704920_220000_/LConn1 -- _CN_275985691_220000_CN_277704920_220000/LConn1
  _CN_312852605_220000_CN_277704920_220000/RConn2 -- T_277704920_220000_/LConn2 -- _CN_275985691_220000_CN_277704920_220000/LConn2
  _CN_312852605_220000_CN_277704920_220000/RConn3 -- T_277704920_220000_/LConn3 -- _CN_275985691_220000_CN_277704920_220000/LConn3 -- bus105/LConn1
  T_147706495_220000_/LConn1 -- _CN_147706495_220000_CN_147708063_220000/RConn1
  T_147706495_220000_/LConn2 -- _CN_147706495_220000_CN_147708063_220000/RConn2
  _CN_147706495_220000_CN_147708063_220000/RConn3 -- T_147706495_220000_/LConn3 -- bus106/LConn1
  T_279711874__/LConn1 -- _CN_279711874_220000_CN_277499262_220000/RConn1
  T_279711874__/LConn2 -- _CN_279711874_220000_CN_277499262_220000/RConn2
  _CN_279711874_220000_CN_277499262_220000/RConn3 -- T_279711874__/LConn3 -- bus107/LConn1
  T_323106340_220000_/LConn1 -- _CN_323106411_220000_CN_323106340_220000/RConn1
  T_323106340_220000_/LConn2 -- _CN_323106411_220000_CN_323106340_220000/RConn2
  _CN_323106411_220000_CN_323106340_220000/RConn3 -- T_323106340_220000_/LConn3 -- bus108/LConn1
  T_277880964__/LConn1 -- _CN_277880964_220000_CN_365843497_220000/LConn1
  T_277880964__/LConn2 -- _CN_277880964_220000_CN_365843497_220000/LConn2
  _CN_277880964_220000_CN_365843497_220000/LConn3 -- T_277880964__/LConn3 -- bus109/LConn1
  _CN_277880964_220000_CN_365843497_220000/RConn1 -- T_365843497__/LConn1 -- _CN_277880965_220000_CN_365843497_220000/RConn1
  _CN_277880964_220000_CN_365843497_220000/RConn2 -- T_365843497__/LConn2 -- _CN_277880965_220000_CN_365843497_220000/RConn2
  _CN_277880964_220000_CN_365843497_220000/RConn3 -- T_365843497__/LConn3 -- _CN_277880965_220000_CN_365843497_220000/RConn3 -- bus110/LConn1
  T_258077674_220000_/LConn1 -- _CN_136348806_220000_CN_258077674_220000/RConn1
  T_258077674_220000_/LConn2 -- _CN_136348806_220000_CN_258077674_220000/RConn2
  _CN_136348806_220000_CN_258077674_220000/RConn3 -- T_258077674_220000_/LConn3 -- bus111/LConn1
  T_279442214__/LConn1 -- _CN_136348806_220000_CN_279442214_220000/RConn1
  T_279442214__/LConn2 -- _CN_136348806_220000_CN_279442214_220000/RConn2
  _CN_136348806_220000_CN_279442214_220000/RConn3 -- T_279442214__/LConn3 -- bus112/LConn1
  _CN_189145223_220000_CN_189139925_220000/LConn1 -- T_189145223_220000_/LConn1 -- _CN_189145223_220000_CN_147708063_220000/RConn1
  _CN_189145223_220000_CN_189139925_220000/LConn2 -- T_189145223_220000_/LConn2 -- _CN_189145223_220000_CN_147708063_220000/RConn2
  _CN_189145223_220000_CN_189139925_220000/LConn3 -- T_189145223_220000_/LConn3 -- _CN_189145223_220000_CN_147708063_220000/RConn3 -- bus113/LConn1
  _CN_189145223_220000_CN_189139925_220000/RConn1 -- T_189139925_220000_/LConn1 -- _CN_147708063_220000_CN_189139925_220000/RConn1
  _CN_189145223_220000_CN_189139925_220000/RConn2 -- T_189139925_220000_/LConn2 -- _CN_147708063_220000_CN_189139925_220000/RConn2
  _CN_189145223_220000_CN_189139925_220000/RConn3 -- T_189139925_220000_/LConn3 -- _CN_147708063_220000_CN_189139925_220000/RConn3 -- bus114/LConn1
  _CN_315303020_220000_CN_178542455_220000/LConn1 -- T_315303020_220000_/LConn1 -- _CN_315303020_220000_CN_383977880_220000/LConn1 -- _CN_315303020_220000_CN_313944391_220000/LConn1
  _CN_315303020_220000_CN_178542455_220000/LConn2 -- T_315303020_220000_/LConn2 -- _CN_315303020_220000_CN_383977880_220000/LConn2 -- _CN_315303020_220000_CN_313944391_220000/LConn2
  _CN_315303020_220000_CN_178542455_220000/LConn3 -- T_315303020_220000_/LConn3 -- _CN_315303020_220000_CN_383977880_220000/LConn3 -- _CN_315303020_220000_CN_313944391_220000/LConn3 -- bus115/LConn1
  _CN_315303020_220000_CN_178542455_220000/RConn1 -- T_178542455_500000_/RConn1 -- _CN_178542455_220000_CN_313944392_220000/LConn1 -- L_178542455/LConn1 -- _CN_178542455_220000_CN_313944391_220000/LConn1
  _CN_315303020_220000_CN_178542455_220000/RConn2 -- T_178542455_500000_/RConn2 -- _CN_178542455_220000_CN_313944392_220000/LConn2 -- L_178542455/LConn2 -- _CN_178542455_220000_CN_313944391_220000/LConn2
  _CN_315303020_220000_CN_178542455_220000/RConn3 -- T_178542455_500000_/RConn3 -- _CN_178542455_220000_CN_313944392_220000/LConn3 -- L_178542455/LConn3 -- bus116/LConn1 -- _CN_178542455_220000_CN_313944391_220000/LConn3
  T_383977880__/LConn1 -- _CN_315303020_220000_CN_383977880_220000/RConn1
  T_383977880__/LConn2 -- _CN_315303020_220000_CN_383977880_220000/RConn2
  _CN_315303020_220000_CN_383977880_220000/RConn3 -- T_383977880__/LConn3 -- bus117/LConn1
  _CN_315303020_220000_CN_313944391_220000/RConn1 -- T_313944391_220000_/LConn1 -- _CN_178542455_220000_CN_313944391_220000/RConn1
  _CN_315303020_220000_CN_313944391_220000/RConn2 -- T_313944391_220000_/LConn2 -- _CN_178542455_220000_CN_313944391_220000/RConn2
  _CN_315303020_220000_CN_313944391_220000/RConn3 -- T_313944391_220000_/LConn3 -- _CN_178542455_220000_CN_313944391_220000/RConn3 -- bus118/LConn1
  _CN_287088780_220000_CN_336382462_220000/LConn1 -- T_287088780_500000_/RConn1 -- L_287088780/LConn1
  _CN_287088780_220000_CN_336382462_220000/LConn2 -- T_287088780_500000_/RConn2 -- L_287088780/LConn2
  _CN_287088780_220000_CN_336382462_220000/LConn3 -- T_287088780_500000_/RConn3 -- L_287088780/LConn3 -- bus119/LConn1
  T_336382462__/LConn1 -- _CN_287088780_220000_CN_336382462_220000/RConn1
  T_336382462__/LConn2 -- _CN_287088780_220000_CN_336382462_220000/RConn2
  _CN_287088780_220000_CN_336382462_220000/RConn3 -- T_336382462__/LConn3 -- bus120/LConn1
  _CN_313934998_220000_CN_384012825_220000/LConn1 -- T_313934998_500000_/RConn1 -- _CN_313934998_220000_CN_314000703_220000/LConn1 -- L_313934998/LConn1
  _CN_313934998_220000_CN_384012825_220000/LConn2 -- T_313934998_500000_/RConn2 -- _CN_313934998_220000_CN_314000703_220000/LConn2 -- L_313934998/LConn2
  _CN_313934998_220000_CN_384012825_220000/LConn3 -- T_313934998_500000_/RConn3 -- _CN_313934998_220000_CN_314000703_220000/LConn3 -- L_313934998/LConn3 -- bus121/LConn1
  T_384012825__/LConn1 -- _CN_313934998_220000_CN_384012825_220000/RConn1
  T_384012825__/LConn2 -- _CN_313934998_220000_CN_384012825_220000/RConn2
  _CN_313934998_220000_CN_384012825_220000/RConn3 -- T_384012825__/LConn3 -- bus122/LConn1
  T_314000703_220000_/LConn1 -- _CN_313934998_220000_CN_314000703_220000/RConn1
  T_314000703_220000_/LConn2 -- _CN_313934998_220000_CN_314000703_220000/RConn2
  _CN_313934998_220000_CN_314000703_220000/RConn3 -- T_314000703_220000_/LConn3 -- bus123/LConn1
  T_160440345__伏陵变电站/LConn1 -- _CN_160440345_220000_CN_286930852_220000/LConn1
  T_160440345__伏陵变电站/LConn2 -- _CN_160440345_220000_CN_286930852_220000/LConn2
  _CN_160440345_220000_CN_286930852_220000/LConn3 -- T_160440345__伏陵变电站/LConn3 -- bus124/LConn1
  _CN_160440345_220000_CN_286930852_220000/RConn1 -- T_286930852__/RConn1 -- _CN_286930852_220000_CN_286930814_220000/LConn1 -- L_286930852/LConn1
  _CN_160440345_220000_CN_286930852_220000/RConn2 -- T_286930852__/RConn2 -- _CN_286930852_220000_CN_286930814_220000/LConn2 -- L_286930852/LConn2
  _CN_160440345_220000_CN_286930852_220000/RConn3 -- T_286930852__/RConn3 -- _CN_286930852_220000_CN_286930814_220000/LConn3 -- L_286930852/LConn3 -- bus125/LConn1
  _CN_275985691_220000_CN_277704920_220000/RConn1 -- T_275985691_500000_房山变电站/RConn1 -- _CN_275985691_220000_CN_279946098_220000/LConn1 -- L_275985691/LConn1
  _CN_275985691_220000_CN_277704920_220000/RConn2 -- T_275985691_500000_房山变电站/RConn2 -- _CN_275985691_220000_CN_279946098_220000/LConn2 -- L_275985691/LConn2
  _CN_275985691_220000_CN_277704920_220000/RConn3 -- T_275985691_500000_房山变电站/RConn3 -- _CN_275985691_220000_CN_279946098_220000/LConn3 -- L_275985691/LConn3 -- bus126/LConn1
  T_279946098__/LConn1 -- _CN_275985691_220000_CN_279946098_220000/RConn1
  T_279946098__/LConn2 -- _CN_275985691_220000_CN_279946098_220000/RConn2
  _CN_275985691_220000_CN_279946098_220000/RConn3 -- T_279946098__/LConn3 -- bus127/LConn1
  T_163162788__/LConn1 -- _CN_163162788_220000_CN_163021047_220000/LConn1
  T_163162788__/LConn2 -- _CN_163162788_220000_CN_163021047_220000/LConn2
  _CN_163162788_220000_CN_163021047_220000/LConn3 -- T_163162788__/LConn3 -- bus128/LConn1
  _CN_163162788_220000_CN_163021047_220000/RConn1 -- T_163021047__/RConn1 -- _CN_163021047_220000_CN_286930805_220000/LConn1 -- L_163021047/LConn1 -- _CN_163162791_220000_CN_163021047_220000/LConn1 -- _CN_163021047_220000_CN_283658122_220000/LConn1 -- _CN_163021047_220000_CN_166670597_220000/LConn1
  _CN_163162788_220000_CN_163021047_220000/RConn2 -- T_163021047__/RConn2 -- _CN_163021047_220000_CN_286930805_220000/LConn2 -- L_163021047/LConn2 -- _CN_163162791_220000_CN_163021047_220000/LConn2 -- _CN_163021047_220000_CN_283658122_220000/LConn2 -- _CN_163021047_220000_CN_166670597_220000/LConn2
  _CN_163162788_220000_CN_163021047_220000/RConn3 -- T_163021047__/RConn3 -- _CN_163021047_220000_CN_286930805_220000/LConn3 -- L_163021047/LConn3 -- bus129/LConn1 -- _CN_163162791_220000_CN_163021047_220000/LConn3 -- _CN_163021047_220000_CN_283658122_220000/LConn3 -- _CN_163021047_220000_CN_166670597_220000/LConn3
  T_163162791__/LConn1 -- _CN_163162791_220000_CN_163021047_220000/RConn1
  T_163162791__/LConn2 -- _CN_163162791_220000_CN_163021047_220000/RConn2
  _CN_163162791_220000_CN_163021047_220000/RConn3 -- T_163162791__/LConn3 -- bus130/LConn1
  T_132503211__/LConn1 -- _CN_132503211_220000_CN_132430137_220000/RConn1
  T_132503211__/LConn2 -- _CN_132503211_220000_CN_132430137_220000/RConn2
  _CN_132503211_220000_CN_132430137_220000/RConn3 -- T_132503211__/LConn3 -- bus131/LConn1
  _CN_128727215_220000_CN_132312011_220000/LConn1 -- T_128727215__/LConn1 -- _CN_128727215_220000_CN_322733769_220000/LConn1
  _CN_128727215_220000_CN_132312011_220000/LConn2 -- T_128727215__/LConn2 -- _CN_128727215_220000_CN_322733769_220000/LConn2
  _CN_128727215_220000_CN_132312011_220000/LConn3 -- T_128727215__/LConn3 -- _CN_128727215_220000_CN_322733769_220000/LConn3 -- bus132/LConn1
  _CN_128727215_220000_CN_132312011_220000/RConn1 -- T_132312011__/LConn1 -- _CN_132430137_220000_CN_132312011_220000/RConn1
  _CN_128727215_220000_CN_132312011_220000/RConn2 -- T_132312011__/LConn2 -- _CN_132430137_220000_CN_132312011_220000/RConn2
  _CN_128727215_220000_CN_132312011_220000/RConn3 -- T_132312011__/LConn3 -- _CN_132430137_220000_CN_132312011_220000/RConn3 -- bus133/LConn1
  T_322733769_220000_/LConn1 -- _CN_128727215_220000_CN_322733769_220000/RConn1
  T_322733769_220000_/LConn2 -- _CN_128727215_220000_CN_322733769_220000/RConn2
  _CN_128727215_220000_CN_322733769_220000/RConn3 -- T_322733769_220000_/LConn3 -- bus134/LConn1
  T_171491187__/LConn1 -- _CN_171491187_220000_CN_132424981_220000/LConn1
  T_171491187__/LConn2 -- _CN_171491187_220000_CN_132424981_220000/LConn2
  _CN_171491187_220000_CN_132424981_220000/LConn3 -- T_171491187__/LConn3 -- bus135/LConn1
  _CN_171491187_220000_CN_132424981_220000/RConn1 -- T_132424981__/RConn1 -- L_132424981/LConn1
  _CN_171491187_220000_CN_132424981_220000/RConn2 -- T_132424981__/RConn2 -- L_132424981/LConn2
  _CN_171491187_220000_CN_132424981_220000/RConn3 -- T_132424981__/RConn3 -- L_132424981/LConn3 -- bus136/LConn1
  _CN_315071509_220000_CN_131286199_220000/LConn1 -- T_315071509_500000_/RConn1 -- L_315071509/LConn1
  _CN_315071509_220000_CN_131286199_220000/LConn2 -- T_315071509_500000_/RConn2 -- L_315071509/LConn2
  _CN_315071509_220000_CN_131286199_220000/LConn3 -- T_315071509_500000_/RConn3 -- L_315071509/LConn3 -- bus137/LConn1
  T_131286199_220000_/LConn1 -- _CN_315071509_220000_CN_131286199_220000/RConn1
  T_131286199_220000_/LConn2 -- _CN_315071509_220000_CN_131286199_220000/RConn2
  _CN_315071509_220000_CN_131286199_220000/RConn3 -- T_131286199_220000_/LConn3 -- bus138/LConn1
  T_171514556_220000_/LConn1 -- _CN_171514556_220000_CN_207327989_220000/LConn1
  T_171514556_220000_/LConn2 -- _CN_171514556_220000_CN_207327989_220000/LConn2
  _CN_171514556_220000_CN_207327989_220000/LConn3 -- T_171514556_220000_/LConn3 -- bus139/LConn1
  _CN_171514556_220000_CN_207327989_220000/RConn1 -- T_207327989_500000_/RConn1 -- L_207327989/LConn1
  _CN_171514556_220000_CN_207327989_220000/RConn2 -- T_207327989_500000_/RConn2 -- L_207327989/LConn2
  _CN_171514556_220000_CN_207327989_220000/RConn3 -- T_207327989_500000_/RConn3 -- L_207327989/LConn3 -- bus140/LConn1
  _CN_279595711_220000_CN_312789337_220000/RConn1 -- T_312789337_220000_/LConn1 -- _CN_312789337_220000_CN_276589719_220000/LConn1
  _CN_279595711_220000_CN_312789337_220000/RConn2 -- T_312789337_220000_/LConn2 -- _CN_312789337_220000_CN_276589719_220000/LConn2
  _CN_279595711_220000_CN_312789337_220000/RConn3 -- T_312789337_220000_/LConn3 -- _CN_312789337_220000_CN_276589719_220000/LConn3 -- bus141/LConn1
  T_170216134__/LConn1 -- _CN_170216134_220000_CN_170206555_220000/RConn1
  T_170216134__/LConn2 -- _CN_170216134_220000_CN_170206555_220000/RConn2
  _CN_170216134_220000_CN_170206555_220000/RConn3 -- T_170216134__/LConn3 -- bus142/LConn1
  T_313944392_220000_/LConn1 -- _CN_178542455_220000_CN_313944392_220000/RConn1
  T_313944392_220000_/LConn2 -- _CN_178542455_220000_CN_313944392_220000/RConn2
  _CN_178542455_220000_CN_313944392_220000/RConn3 -- T_313944392_220000_/LConn3 -- bus143/LConn1
  T_313672407_500000_/LConn1 -- _CN_313672407_220000_CN_166670643_220000/LConn1
  T_313672407_500000_/LConn2 -- _CN_313672407_220000_CN_166670643_220000/LConn2
  _CN_313672407_220000_CN_166670643_220000/LConn3 -- T_313672407_500000_/LConn3 -- bus144/LConn1
  _CN_313672407_220000_CN_166670643_220000/RConn1 -- T_166670643__/LConn1 -- _CN_166670643_220000_CN_166785367_220000/LConn1 -- _CN_166670641_220000_CN_166670643_220000/LConn1
  _CN_313672407_220000_CN_166670643_220000/RConn2 -- T_166670643__/LConn2 -- _CN_166670643_220000_CN_166785367_220000/LConn2 -- _CN_166670641_220000_CN_166670643_220000/LConn2
  _CN_313672407_220000_CN_166670643_220000/RConn3 -- T_166670643__/LConn3 -- _CN_166670643_220000_CN_166785367_220000/LConn3 -- bus145/LConn1 -- _CN_166670641_220000_CN_166670643_220000/LConn3
  T_280819419__/LConn1 -- _CN_280819419_220000_CN_181221620_220000/LConn1
  T_280819419__/LConn2 -- _CN_280819419_220000_CN_181221620_220000/LConn2
  _CN_280819419_220000_CN_181221620_220000/LConn3 -- T_280819419__/LConn3 -- bus146/LConn1
  _CN_280819419_220000_CN_181221620_220000/RConn1 -- T_181221620_500000_500KV三汊湾变电站/RConn1 -- L_181221620/LConn1
  _CN_280819419_220000_CN_181221620_220000/RConn2 -- T_181221620_500000_500KV三汊湾变电站/RConn2 -- L_181221620/LConn2
  _CN_280819419_220000_CN_181221620_220000/RConn3 -- T_181221620_500000_500KV三汊湾变电站/RConn3 -- L_181221620/LConn3 -- bus147/LConn1
  _CN_145499358_220000_CN_121056862_220000/RConn1 -- G_121056862_/RConn1 -- _CN_105834287_220000_CN_121056862_220000/LConn1 -- _CN_283658133_500000_CN_121056862_220000/LConn1
  _CN_145499358_220000_CN_121056862_220000/RConn2 -- G_121056862_/RConn2 -- _CN_105834287_220000_CN_121056862_220000/LConn2 -- _CN_283658133_500000_CN_121056862_220000/LConn2
  _CN_145499358_220000_CN_121056862_220000/RConn3 -- G_121056862_/RConn3 -- _CN_105834287_220000_CN_121056862_220000/LConn3 -- _CN_283658133_500000_CN_121056862_220000/LConn3 -- bus148/LConn1
  T_287236840__/LConn1 -- _CN_287236840_220000_CN_166670597_220000/LConn1
  T_287236840__/LConn2 -- _CN_287236840_220000_CN_166670597_220000/LConn2
  _CN_287236840_220000_CN_166670597_220000/LConn3 -- T_287236840__/LConn3 -- bus149/LConn1
  _CN_287236840_220000_CN_166670597_220000/RConn1 -- T_166670597__/RConn1 -- _CN_163021047_220000_CN_166670597_220000/RConn1 -- L_166670597/LConn1
  _CN_287236840_220000_CN_166670597_220000/RConn2 -- T_166670597__/RConn2 -- _CN_163021047_220000_CN_166670597_220000/RConn2 -- L_166670597/LConn2
  _CN_287236840_220000_CN_166670597_220000/RConn3 -- T_166670597__/RConn3 -- _CN_163021047_220000_CN_166670597_220000/RConn3 -- L_166670597/LConn3 -- bus150/LConn1
  T_287236841__/LConn1 -- _CN_287236841_220000_CN_104955692_220000/LConn1
  T_287236841__/LConn2 -- _CN_287236841_220000_CN_104955692_220000/LConn2
  _CN_287236841_220000_CN_104955692_220000/LConn3 -- T_287236841__/LConn3 -- bus151/LConn1
  _CN_287236841_220000_CN_104955692_220000/RConn1 -- T_104955692_220000_/LConn1 -- _CN_104955692_220000_CN_105834291_220000/LConn1 -- _CN_104955692_220000_CN_106027361_220000/LConn1 -- _CN_106027267_220000_CN_104955692_220000/LConn1
  _CN_287236841_220000_CN_104955692_220000/RConn2 -- T_104955692_220000_/LConn2 -- _CN_104955692_220000_CN_105834291_220000/LConn2 -- _CN_104955692_220000_CN_106027361_220000/LConn2 -- _CN_106027267_220000_CN_104955692_220000/LConn2
  _CN_287236841_220000_CN_104955692_220000/RConn3 -- T_104955692_220000_/LConn3 -- _CN_104955692_220000_CN_105834291_220000/LConn3 -- _CN_104955692_220000_CN_106027361_220000/LConn3 -- bus152/LConn1 -- _CN_106027267_220000_CN_104955692_220000/LConn3
  T_170703091__/LConn1 -- _CN_170703091_220000_CN_170703096_220000/LConn1
  T_170703091__/LConn2 -- _CN_170703091_220000_CN_170703096_220000/LConn2
  _CN_170703091_220000_CN_170703096_220000/LConn3 -- T_170703091__/LConn3 -- bus153/LConn1
  _CN_170703091_220000_CN_170703096_220000/RConn1 -- T_170703096_500000_/RConn1 -- _CN_170703094_220000_CN_170703096_220000/LConn1 -- L_170703096/LConn1
  _CN_170703091_220000_CN_170703096_220000/RConn2 -- T_170703096_500000_/RConn2 -- _CN_170703094_220000_CN_170703096_220000/LConn2 -- L_170703096/LConn2
  _CN_170703091_220000_CN_170703096_220000/RConn3 -- T_170703096_500000_/RConn3 -- _CN_170703094_220000_CN_170703096_220000/LConn3 -- L_170703096/LConn3 -- bus154/LConn1
  T_170703094_220000_/LConn1 -- _CN_170703094_220000_CN_170703096_220000/RConn1
  T_170703094_220000_/LConn2 -- _CN_170703094_220000_CN_170703096_220000/RConn2
  _CN_170703094_220000_CN_170703096_220000/RConn3 -- T_170703094_220000_/LConn3 -- bus155/LConn1
  _CN_163021047_220000_CN_283658122_220000/RConn1 -- T_283658122__/LConn1 -- _CN_284083293_220000_CN_283658122_220000/RConn1
  _CN_163021047_220000_CN_283658122_220000/RConn2 -- T_283658122__/LConn2 -- _CN_284083293_220000_CN_283658122_220000/RConn2
  _CN_163021047_220000_CN_283658122_220000/RConn3 -- T_283658122__/LConn3 -- _CN_284083293_220000_CN_283658122_220000/RConn3 -- bus156/LConn1
  T_286930805__/LConn1 -- _CN_163021047_220000_CN_286930805_220000/RConn1
  T_286930805__/LConn2 -- _CN_163021047_220000_CN_286930805_220000/RConn2
  _CN_163021047_220000_CN_286930805_220000/RConn3 -- T_286930805__/LConn3 -- bus157/LConn1
  T_132428536_220000_/LConn1 -- _CN_132428536_220000_CN_132312010_220000/LConn1
  T_132428536_220000_/LConn2 -- _CN_132428536_220000_CN_132312010_220000/LConn2
  _CN_132428536_220000_CN_132312010_220000/LConn3 -- T_132428536_220000_/LConn3 -- bus158/LConn1
  _CN_132428536_220000_CN_132312010_220000/RConn1 -- T_132312010_500000_/LConn1 -- _CN_132430137_220000_CN_132312010_220000/RConn1 -- _CN_128731545_220000_CN_132312010_220000/LConn1 -- _CN_132311997_220000_CN_132312010_220000/LConn1
  _CN_132428536_220000_CN_132312010_220000/RConn2 -- T_132312010_500000_/LConn2 -- _CN_132430137_220000_CN_132312010_220000/RConn2 -- _CN_128731545_220000_CN_132312010_220000/LConn2 -- _CN_132311997_220000_CN_132312010_220000/LConn2
  _CN_132428536_220000_CN_132312010_220000/RConn3 -- T_132312010_500000_/LConn3 -- _CN_132430137_220000_CN_132312010_220000/RConn3 -- _CN_128731545_220000_CN_132312010_220000/LConn3 -- _CN_132311997_220000_CN_132312010_220000/LConn3 -- bus159/LConn1
  T_333873642_220000_/LConn1 -- _CN_333873642_220000_CN_333873652_220000/LConn1
  T_333873642_220000_/LConn2 -- _CN_333873642_220000_CN_333873652_220000/LConn2
  _CN_333873642_220000_CN_333873652_220000/LConn3 -- T_333873642_220000_/LConn3 -- bus160/LConn1
  T_333873652_500000_/LConn1 -- _CN_333873642_220000_CN_333873652_220000/RConn1
  T_333873652_500000_/LConn2 -- _CN_333873642_220000_CN_333873652_220000/RConn2
  _CN_333873642_220000_CN_333873652_220000/RConn3 -- T_333873652_500000_/LConn3 -- bus161/LConn1
  T_95801089__/LConn1 -- _CN_95801089_220000_CN_95805677_220000/RConn1
  T_95801089__/LConn2 -- _CN_95801089_220000_CN_95805677_220000/RConn2
  _CN_95801089_220000_CN_95805677_220000/RConn3 -- T_95801089__/LConn3 -- bus162/LConn1
  _CN_106027267_220000_CN_106027361_220000/LConn1 -- T_106027267_220000_/LConn1 -- _CN_106027267_220000_CN_104955692_220000/RConn1
  _CN_106027267_220000_CN_106027361_220000/LConn2 -- T_106027267_220000_/LConn2 -- _CN_106027267_220000_CN_104955692_220000/RConn2
  _CN_106027267_220000_CN_106027361_220000/LConn3 -- T_106027267_220000_/LConn3 -- _CN_106027267_220000_CN_104955692_220000/RConn3 -- bus163/LConn1
  _CN_106027267_220000_CN_106027361_220000/RConn1 -- T_106027361_220000_/LConn1 -- _CN_104955692_220000_CN_106027361_220000/RConn1
  _CN_106027267_220000_CN_106027361_220000/RConn2 -- T_106027361_220000_/LConn2 -- _CN_104955692_220000_CN_106027361_220000/RConn2
  _CN_106027267_220000_CN_106027361_220000/RConn3 -- T_106027361_220000_/LConn3 -- _CN_104955692_220000_CN_106027361_220000/RConn3 -- bus164/LConn1
  T_321557804_220000_/LConn1 -- _CN_321557804_220000_CN_133523400_220000/RConn1
  T_321557804_220000_/LConn2 -- _CN_321557804_220000_CN_133523400_220000/RConn2
  _CN_321557804_220000_CN_133523400_220000/RConn3 -- T_321557804_220000_/LConn3 -- bus165/LConn1
  T_314893527_220000_/LConn1 -- _CN_314893527_220000_CN_314883039_220000/LConn1
  T_314893527_220000_/LConn2 -- _CN_314893527_220000_CN_314883039_220000/LConn2
  _CN_314893527_220000_CN_314883039_220000/LConn3 -- T_314893527_220000_/LConn3 -- bus166/LConn1
  _CN_314893527_220000_CN_314883039_220000/RConn1 -- T_314883039_500000_/RConn1 -- L_314883039/LConn1
  _CN_314893527_220000_CN_314883039_220000/RConn2 -- T_314883039_500000_/RConn2 -- L_314883039/LConn2
  _CN_314893527_220000_CN_314883039_220000/RConn3 -- T_314883039_500000_/RConn3 -- L_314883039/LConn3 -- bus167/LConn1
  T_105894253__/LConn1 -- _CN_104955669_220000_CN_105894253_220000/RConn1
  T_105894253__/LConn2 -- _CN_104955669_220000_CN_105894253_220000/RConn2
  _CN_104955669_220000_CN_105894253_220000/RConn3 -- T_105894253__/LConn3 -- bus168/LConn1
  T_312588761_220000_/LConn1 -- _CN_312588761_220000_CN_312588760_220000/LConn1
  T_312588761_220000_/LConn2 -- _CN_312588761_220000_CN_312588760_220000/LConn2
  _CN_312588761_220000_CN_312588760_220000/LConn3 -- T_312588761_220000_/LConn3 -- bus169/LConn1
  _CN_312588761_220000_CN_312588760_220000/RConn1 -- T_312588760_500000_/RConn1 -- L_312588760/LConn1
  _CN_312588761_220000_CN_312588760_220000/RConn2 -- T_312588760_500000_/RConn2 -- L_312588760/LConn2
  _CN_312588761_220000_CN_312588760_220000/RConn3 -- T_312588760_500000_/RConn3 -- L_312588760/LConn3 -- bus170/LConn1
  _CN_151766812_220000_CN_322733771_220000/LConn1 -- T_151766812_500000;220000_/RConn1 -- L_151766812/LConn1
  _CN_151766812_220000_CN_322733771_220000/LConn2 -- T_151766812_500000;220000_/RConn2 -- L_151766812/LConn2
  _CN_151766812_220000_CN_322733771_220000/LConn3 -- T_151766812_500000;220000_/RConn3 -- L_151766812/LConn3 -- bus171/LConn1
  T_322733771__/LConn1 -- _CN_151766812_220000_CN_322733771_220000/RConn1
  T_322733771__/LConn2 -- _CN_151766812_220000_CN_322733771_220000/RConn2
  _CN_151766812_220000_CN_322733771_220000/RConn3 -- T_322733771__/LConn3 -- bus172/LConn1
  T_166670641__/LConn1 -- _CN_166670641_220000_CN_166670643_220000/RConn1
  T_166670641__/LConn2 -- _CN_166670641_220000_CN_166670643_220000/RConn2
  _CN_166670641_220000_CN_166670643_220000/RConn3 -- T_166670641__/LConn3 -- bus173/LConn1
  T_329740587_500000_/LConn1 -- _CN_329740587_220000_CN_149239742_220000/LConn1
  T_329740587_500000_/LConn2 -- _CN_329740587_220000_CN_149239742_220000/LConn2
  _CN_329740587_220000_CN_149239742_220000/LConn3 -- T_329740587_500000_/LConn3 -- bus174/LConn1
  T_149239742_220000_/LConn1 -- _CN_329740587_220000_CN_149239742_220000/RConn1
  T_149239742_220000_/LConn2 -- _CN_329740587_220000_CN_149239742_220000/RConn2
  _CN_329740587_220000_CN_149239742_220000/RConn3 -- T_149239742_220000_/LConn3 -- bus175/LConn1
  G_105834291_/RConn1 -- _CN_104955692_220000_CN_105834291_220000/RConn1
  G_105834291_/RConn2 -- _CN_104955692_220000_CN_105834291_220000/RConn2
  _CN_104955692_220000_CN_105834291_220000/RConn3 -- G_105834291_/RConn3 -- bus176/LConn1
  T_166670638__/LConn1 -- _CN_166670638_220000_CN_166785368_220000/LConn1
